simulink model "gravcomp"  (Simulink 7.5)
settings: Solver=ode3  StartTime=0.0  StopTime=inf  FixedStep=.002  RelTol=1e-3
values from neighbouring files (symbols this model uses):
  arm_home = [ -0.1106   -1.9490   -0.1920    3.1840 ]    [NEW_PID_4DOF.m]    (also in SetPoint_Control.m = [ -0.1106   -1.9490   -0.1920    3.1840    0.2825    0.0969 ; Stochastic_coriolis.m = [  -0.1106   -1.9490   -0.1920    3.1840    0.2825    0.0969; Untitled4.m = [ -0.1106   -1.9490   -0.1920    3.1840    0.2825    0.0969 )
undefined symbols (not defined in the file or in its folder): arm_j2mt, arm_m2jp, bit, CAN_init, enc_per_rev, fdesignblkfcn, FT_init, gcbh, hand_on, MT_init, puck_I_per_Nm, rotFT2Hand, sample_time, Standard, VL1_init, VL2_init
libraries: simulink x358, xpclib x28, xpcutilitieslib x6, dspmathops x1
(part 2 of 3)

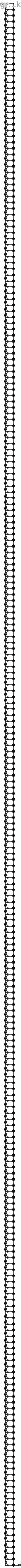
== system gravcomp/Get FT/Get Force Torque/New Filter/Generated Filter Block ==
  Input : Inport
  BodyDelay{2..260} (259 alike) : simulink/Discrete/Integer Delay  vinit=0  samptime=-1  NumDelays=1
  BodyLSum{2..260} (259 alike) : Sum  Inputs=++|  OutScaling=1  RndMeth=Nearest  SaturateOnIntegerOverflow=on  OutDataTypeStr=Inherit: Same as first input
  b(1) : Gain  Gain=0.00070417510961843762  ParameterDataTypeMode=Specify via dialog  ParameterDataType=float('double')  ParamDataTypeStr=float('double')  OutScaling=1  RndMeth=Nearest  SaturateOnIntegerOverflow=on  OutDataTypeStr=Inherit: Same as input
  b(10) : Gain  Gain=0.00065890295760926093  ParameterDataTypeMode=Specify via dialog  ParameterDataType=float('double')  ParamDataTypeStr=float('double')  OutScaling=1  RndMeth=Nearest  SaturateOnIntegerOverflow=on  OutDataTypeStr=Inherit: Same as input
  b(100) : Gain  Gain=0.0062955708769956709  ParameterDataTypeMode=Specify via dialog  ParameterDataType=float('double')  ParamDataTypeStr=float('double')  OutScaling=1  RndMeth=Nearest  SaturateOnIntegerOverflow=on  OutDataTypeStr=Inherit: Same as input
  b(101) : Gain  Gain=0.0071285779409714038  ParameterDataTypeMode=Specify via dialog  ParameterDataType=float('double')  ParamDataTypeStr=float('double')  OutScaling=1  RndMeth=Nearest  SaturateOnIntegerOverflow=on  OutDataTypeStr=Inherit: Same as input
  b(102) : Gain  Gain=0.0079758397591894736  ParameterDataTypeMode=Specify via dialog  ParameterDataType=float('double')  ParamDataTypeStr=float('double')  OutScaling=1  RndMeth=Nearest  SaturateOnIntegerOverflow=on  OutDataTypeStr=Inherit: Same as input
  b(103) : Gain  Gain=0.0088344622316554079  ParameterDataTypeMode=Specify via dialog  ParameterDataType=float('double')  ParamDataTypeStr=float('double')  OutScaling=1  RndMeth=Nearest  SaturateOnIntegerOverflow=on  OutDataTypeStr=Inherit: Same as input
  b(104) : Gain  Gain=0.0097014714889568053  ParameterDataTypeMode=Specify via dialog  ParameterDataType=float('double')  ParamDataTypeStr=float('double')  OutScaling=1  RndMeth=Nearest  SaturateOnIntegerOverflow=on  OutDataTypeStr=Inherit: Same as input
  b(105) : Gain  Gain=0.010573811729065394  ParameterDataTypeMode=Specify via dialog  ParameterDataType=float('double')  ParamDataTypeStr=float('double')  OutScaling=1  RndMeth=Nearest  SaturateOnIntegerOverflow=on  OutDataTypeStr=Inherit: Same as input
  b(106) : Gain  Gain=0.011448280041578808  ParameterDataTypeMode=Specify via dialog  ParameterDataType=float('double')  ParamDataTypeStr=float('double')  OutScaling=1  RndMeth=Nearest  SaturateOnIntegerOverflow=on  OutDataTypeStr=Inherit: Same as input
  b(107) : Gain  Gain=0.012321705260453951  ParameterDataTypeMode=Specify via dialog  ParameterDataType=float('double')  ParamDataTypeStr=float('double')  OutScaling=1  RndMeth=Nearest  SaturateOnIntegerOverflow=on  OutDataTypeStr=Inherit: Same as input
  b(108) : Gain  Gain=0.01319080449047489  ParameterDataTypeMode=Specify via dialog  ParameterDataType=float('double')  ParamDataTypeStr=float('double')  OutScaling=1  RndMeth=Nearest  SaturateOnIntegerOverflow=on  OutDataTypeStr=Inherit: Same as input
  b(109) : Gain  Gain=0.014052286654709126  ParameterDataTypeMode=Specify via dialog  ParameterDataType=float('double')  ParamDataTypeStr=float('double')  OutScaling=1  RndMeth=Nearest  SaturateOnIntegerOverflow=on  OutDataTypeStr=Inherit: Same as input
  b(11) : Gain  Gain=0.00072315700075571872  ParameterDataTypeMode=Specify via dialog  ParameterDataType=float('double')  ParamDataTypeStr=float('double')  OutScaling=1  RndMeth=Nearest  SaturateOnIntegerOverflow=on  OutDataTypeStr=Inherit: Same as input
  b(110) : Gain  Gain=0.014902829506351663  ParameterDataTypeMode=Specify via dialog  ParameterDataType=float('double')  ParamDataTypeStr=float('double')  OutScaling=1  RndMeth=Nearest  SaturateOnIntegerOverflow=on  OutDataTypeStr=Inherit: Same as input
  b(111) : Gain  Gain=0.015739153848427601  ParameterDataTypeMode=Specify via dialog  ParameterDataType=float('double')  ParamDataTypeStr=float('double')  OutScaling=1  RndMeth=Nearest  SaturateOnIntegerOverflow=on  OutDataTypeStr=Inherit: Same as input
  b(112) : Gain  Gain=0.016557936832079102  ParameterDataTypeMode=Specify via dialog  ParameterDataType=float('double')  ParamDataTypeStr=float('double')  OutScaling=1  RndMeth=Nearest  SaturateOnIntegerOverflow=on  OutDataTypeStr=Inherit: Same as input
  b(113) : Gain  Gain=0.017355946398475892  ParameterDataTypeMode=Specify via dialog  ParameterDataType=float('double')  ParamDataTypeStr=float('double')  OutScaling=1  RndMeth=Nearest  SaturateOnIntegerOverflow=on  OutDataTypeStr=Inherit: Same as input
  b(114) : Gain  Gain=0.018129972748423043  ParameterDataTypeMode=Specify via dialog  ParameterDataType=float('double')  ParamDataTypeStr=float('double')  OutScaling=1  RndMeth=Nearest  SaturateOnIntegerOverflow=on  OutDataTypeStr=Inherit: Same as input
  b(115) : Gain  Gain=0.018876872775595334  ParameterDataTypeMode=Specify via dialog  ParameterDataType=float('double')  ParamDataTypeStr=float('double')  OutScaling=1  RndMeth=Nearest  SaturateOnIntegerOverflow=on  OutDataTypeStr=Inherit: Same as input
  b(116) : Gain  Gain=0.01959360140160285  ParameterDataTypeMode=Specify via dialog  ParameterDataType=float('double')  ParamDataTypeStr=float('double')  OutScaling=1  RndMeth=Nearest  SaturateOnIntegerOverflow=on  OutDataTypeStr=Inherit: Same as input
  b(117) : Gain  Gain=0.02027722646982065  ParameterDataTypeMode=Specify via dialog  ParameterDataType=float('double')  ParamDataTypeStr=float('double')  OutScaling=1  RndMeth=Nearest  SaturateOnIntegerOverflow=on  OutDataTypeStr=Inherit: Same as input
  b(118) : Gain  Gain=0.020924875790597104  ParameterDataTypeMode=Specify via dialog  ParameterDataType=float('double')  ParamDataTypeStr=float('double')  OutScaling=1  RndMeth=Nearest  SaturateOnIntegerOverflow=on  OutDataTypeStr=Inherit: Same as input
  b(119) : Gain  Gain=0.021533887742310798  ParameterDataTypeMode=Specify via dialog  ParameterDataType=float('double')  ParamDataTypeStr=float('double')  OutScaling=1  RndMeth=Nearest  SaturateOnIntegerOverflow=on  OutDataTypeStr=Inherit: Same as input
  b(12) : Gain  Gain=0.00078945898775655888  ParameterDataTypeMode=Specify via dialog  ParameterDataType=float('double')  ParamDataTypeStr=float('double')  OutScaling=1  RndMeth=Nearest  SaturateOnIntegerOverflow=on  OutDataTypeStr=Inherit: Same as input
  b(120) : Gain  Gain=0.022101695679814737  ParameterDataTypeMode=Specify via dialog  ParameterDataType=float('double')  ParamDataTypeStr=float('double')  OutScaling=1  RndMeth=Nearest  SaturateOnIntegerOverflow=on  OutDataTypeStr=Inherit: Same as input
  b(121) : Gain  Gain=0.022625902042927921  ParameterDataTypeMode=Specify via dialog  ParameterDataType=float('double')  ParamDataTypeStr=float('double')  OutScaling=1  RndMeth=Nearest  SaturateOnIntegerOverflow=on  OutDataTypeStr=Inherit: Same as input
  b(122) : Gain  Gain=0.023104290316677902  ParameterDataTypeMode=Specify via dialog  ParameterDataType=float('double')  ParamDataTypeStr=float('double')  OutScaling=1  RndMeth=Nearest  SaturateOnIntegerOverflow=on  OutDataTypeStr=Inherit: Same as input
  b(123) : Gain  Gain=0.023534842993415066  ParameterDataTypeMode=Specify via dialog  ParameterDataType=float('double')  ParamDataTypeStr=float('double')  OutScaling=1  RndMeth=Nearest  SaturateOnIntegerOverflow=on  OutDataTypeStr=Inherit: Same as input
  b(124) : Gain  Gain=0.023915699194656088  ParameterDataTypeMode=Specify via dialog  ParameterDataType=float('double')  ParamDataTypeStr=float('double')  OutScaling=1  RndMeth=Nearest  SaturateOnIntegerOverflow=on  OutDataTypeStr=Inherit: Same as input
  b(125) : Gain  Gain=0.024245248888987846  ParameterDataTypeMode=Specify via dialog  ParameterDataType=float('double')  ParamDataTypeStr=float('double')  OutScaling=1  RndMeth=Nearest  SaturateOnIntegerOverflow=on  OutDataTypeStr=Inherit: Same as input
  b(126) : Gain  Gain=0.024522074604789321  ParameterDataTypeMode=Specify via dialog  ParameterDataType=float('double')  ParamDataTypeStr=float('double')  OutScaling=1  RndMeth=Nearest  SaturateOnIntegerOverflow=on  OutDataTypeStr=Inherit: Same as input
  b(127) : Gain  Gain=0.024744974417626367  ParameterDataTypeMode=Specify via dialog  ParameterDataType=float('double')  ParamDataTypeStr=float('double')  OutScaling=1  RndMeth=Nearest  SaturateOnIntegerOverflow=on  OutDataTypeStr=Inherit: Same as input
  b(128) : Gain  Gain=0.024913000551013219  ParameterDataTypeMode=Specify via dialog  ParameterDataType=float('double')  ParamDataTypeStr=float('double')  OutScaling=1  RndMeth=Nearest  SaturateOnIntegerOverflow=on  OutDataTypeStr=Inherit: Same as input
  b(129) : Gain  Gain=0.025025430343517754  ParameterDataTypeMode=Specify via dialog  ParameterDataType=float('double')  ParamDataTypeStr=float('double')  OutScaling=1  RndMeth=Nearest  SaturateOnIntegerOverflow=on  OutDataTypeStr=Inherit: Same as input
  b(13) : Gain  Gain=0.00085906126191019659  ParameterDataTypeMode=Specify via dialog  ParameterDataType=float('double')  ParamDataTypeStr=float('double')  OutScaling=1  RndMeth=Nearest  SaturateOnIntegerOverflow=on  OutDataTypeStr=Inherit: Same as input
  b(130) : Gain  Gain=0.025081755990063945  ParameterDataTypeMode=Specify via dialog  ParameterDataType=float('double')  ParamDataTypeStr=float('double')  OutScaling=1  RndMeth=Nearest  SaturateOnIntegerOverflow=on  OutDataTypeStr=Inherit: Same as input
  b(131) : Gain  Gain=0.025081755990063945  ParameterDataTypeMode=Specify via dialog  ParameterDataType=float('double')  ParamDataTypeStr=float('double')  OutScaling=1  RndMeth=Nearest  SaturateOnIntegerOverflow=on  OutDataTypeStr=Inherit: Same as input
  b(132) : Gain  Gain=0.025025430343517754  ParameterDataTypeMode=Specify via dialog  ParameterDataType=float('double')  ParamDataTypeStr=float('double')  OutScaling=1  RndMeth=Nearest  SaturateOnIntegerOverflow=on  OutDataTypeStr=Inherit: Same as input
  b(133) : Gain  Gain=0.024913000551013219  ParameterDataTypeMode=Specify via dialog  ParameterDataType=float('double')  ParamDataTypeStr=float('double')  OutScaling=1  RndMeth=Nearest  SaturateOnIntegerOverflow=on  OutDataTypeStr=Inherit: Same as input
  b(134) : Gain  Gain=0.024744974417626367  ParameterDataTypeMode=Specify via dialog  ParameterDataType=float('double')  ParamDataTypeStr=float('double')  OutScaling=1  RndMeth=Nearest  SaturateOnIntegerOverflow=on  OutDataTypeStr=Inherit: Same as input
  b(135) : Gain  Gain=0.024522074604789321  ParameterDataTypeMode=Specify via dialog  ParameterDataType=float('double')  ParamDataTypeStr=float('double')  OutScaling=1  RndMeth=Nearest  SaturateOnIntegerOverflow=on  OutDataTypeStr=Inherit: Same as input
  b(136) : Gain  Gain=0.024245248888987846  ParameterDataTypeMode=Specify via dialog  ParameterDataType=float('double')  ParamDataTypeStr=float('double')  OutScaling=1  RndMeth=Nearest  SaturateOnIntegerOverflow=on  OutDataTypeStr=Inherit: Same as input
  b(137) : Gain  Gain=0.023915699194656088  ParameterDataTypeMode=Specify via dialog  ParameterDataType=float('double')  ParamDataTypeStr=float('double')  OutScaling=1  RndMeth=Nearest  SaturateOnIntegerOverflow=on  OutDataTypeStr=Inherit: Same as input
  b(138) : Gain  Gain=0.023534842993415066  ParameterDataTypeMode=Specify via dialog  ParameterDataType=float('double')  ParamDataTypeStr=float('double')  OutScaling=1  RndMeth=Nearest  SaturateOnIntegerOverflow=on  OutDataTypeStr=Inherit: Same as input
  b(139) : Gain  Gain=0.023104290316677902  ParameterDataTypeMode=Specify via dialog  ParameterDataType=float('double')  ParamDataTypeStr=float('double')  OutScaling=1  RndMeth=Nearest  SaturateOnIntegerOverflow=on  OutDataTypeStr=Inherit: Same as input
  b(14) : Gain  Gain=0.000928205688470267  ParameterDataTypeMode=Specify via dialog  ParameterDataType=float('double')  ParamDataTypeStr=float('double')  OutScaling=1  RndMeth=Nearest  SaturateOnIntegerOverflow=on  OutDataTypeStr=Inherit: Same as input
  b(140) : Gain  Gain=0.022625902042927921  ParameterDataTypeMode=Specify via dialog  ParameterDataType=float('double')  ParamDataTypeStr=float('double')  OutScaling=1  RndMeth=Nearest  SaturateOnIntegerOverflow=on  OutDataTypeStr=Inherit: Same as input
  b(141) : Gain  Gain=0.022101695679814737  ParameterDataTypeMode=Specify via dialog  ParameterDataType=float('double')  ParamDataTypeStr=float('double')  OutScaling=1  RndMeth=Nearest  SaturateOnIntegerOverflow=on  OutDataTypeStr=Inherit: Same as input
  b(142) : Gain  Gain=0.021533887742310798  ParameterDataTypeMode=Specify via dialog  ParameterDataType=float('double')  ParamDataTypeStr=float('double')  OutScaling=1  RndMeth=Nearest  SaturateOnIntegerOverflow=on  OutDataTypeStr=Inherit: Same as input
  b(143) : Gain  Gain=0.020924875790597104  ParameterDataTypeMode=Specify via dialog  ParameterDataType=float('double')  ParamDataTypeStr=float('double')  OutScaling=1  RndMeth=Nearest  SaturateOnIntegerOverflow=on  OutDataTypeStr=Inherit: Same as input
  b(144) : Gain  Gain=0.02027722646982065  ParameterDataTypeMode=Specify via dialog  ParameterDataType=float('double')  ParamDataTypeStr=float('double')  OutScaling=1  RndMeth=Nearest  SaturateOnIntegerOverflow=on  OutDataTypeStr=Inherit: Same as input
  b(145) : Gain  Gain=0.01959360140160285  ParameterDataTypeMode=Specify via dialog  ParameterDataType=float('double')  ParamDataTypeStr=float('double')  OutScaling=1  RndMeth=Nearest  SaturateOnIntegerOverflow=on  OutDataTypeStr=Inherit: Same as input
  b(146) : Gain  Gain=0.018876872775595334  ParameterDataTypeMode=Specify via dialog  ParameterDataType=float('double')  ParamDataTypeStr=float('double')  OutScaling=1  RndMeth=Nearest  SaturateOnIntegerOverflow=on  OutDataTypeStr=Inherit: Same as input
  b(147) : Gain  Gain=0.018129972748423043  ParameterDataTypeMode=Specify via dialog  ParameterDataType=float('double')  ParamDataTypeStr=float('double')  OutScaling=1  RndMeth=Nearest  SaturateOnIntegerOverflow=on  OutDataTypeStr=Inherit: Same as input
  b(148) : Gain  Gain=0.017355946398475892  ParameterDataTypeMode=Specify via dialog  ParameterDataType=float('double')  ParamDataTypeStr=float('double')  OutScaling=1  RndMeth=Nearest  SaturateOnIntegerOverflow=on  OutDataTypeStr=Inherit: Same as input
  b(149) : Gain  Gain=0.016557936832079102  ParameterDataTypeMode=Specify via dialog  ParameterDataType=float('double')  ParamDataTypeStr=float('double')  OutScaling=1  RndMeth=Nearest  SaturateOnIntegerOverflow=on  OutDataTypeStr=Inherit: Same as input
  b(15) : Gain  Gain=0.00099957917679242272  ParameterDataTypeMode=Specify via dialog  ParameterDataType=float('double')  ParamDataTypeStr=float('double')  OutScaling=1  RndMeth=Nearest  SaturateOnIntegerOverflow=on  OutDataTypeStr=Inherit: Same as input
  b(150) : Gain  Gain=0.015739153848427601  ParameterDataTypeMode=Specify via dialog  ParameterDataType=float('double')  ParamDataTypeStr=float('double')  OutScaling=1  RndMeth=Nearest  SaturateOnIntegerOverflow=on  OutDataTypeStr=Inherit: Same as input
  b(151) : Gain  Gain=0.014902829506351663  ParameterDataTypeMode=Specify via dialog  ParameterDataType=float('double')  ParamDataTypeStr=float('double')  OutScaling=1  RndMeth=Nearest  SaturateOnIntegerOverflow=on  OutDataTypeStr=Inherit: Same as input
  b(152) : Gain  Gain=0.014052286654709126  ParameterDataTypeMode=Specify via dialog  ParameterDataType=float('double')  ParamDataTypeStr=float('double')  OutScaling=1  RndMeth=Nearest  SaturateOnIntegerOverflow=on  OutDataTypeStr=Inherit: Same as input
  b(153) : Gain  Gain=0.01319080449047489  ParameterDataTypeMode=Specify via dialog  ParameterDataType=float('double')  ParamDataTypeStr=float('double')  OutScaling=1  RndMeth=Nearest  SaturateOnIntegerOverflow=on  OutDataTypeStr=Inherit: Same as input
  b(154) : Gain  Gain=0.012321705260453951  ParameterDataTypeMode=Specify via dialog  ParameterDataType=float('double')  ParamDataTypeStr=float('double')  OutScaling=1  RndMeth=Nearest  SaturateOnIntegerOverflow=on  OutDataTypeStr=Inherit: Same as input
  b(155) : Gain  Gain=0.011448280041578808  ParameterDataTypeMode=Specify via dialog  ParameterDataType=float('double')  ParamDataTypeStr=float('double')  OutScaling=1  RndMeth=Nearest  SaturateOnIntegerOverflow=on  OutDataTypeStr=Inherit: Same as input
  b(156) : Gain  Gain=0.010573811729065394  ParameterDataTypeMode=Specify via dialog  ParameterDataType=float('double')  ParamDataTypeStr=float('double')  OutScaling=1  RndMeth=Nearest  SaturateOnIntegerOverflow=on  OutDataTypeStr=Inherit: Same as input
  b(157) : Gain  Gain=0.0097014714889568053  ParameterDataTypeMode=Specify via dialog  ParameterDataType=float('double')  ParamDataTypeStr=float('double')  OutScaling=1  RndMeth=Nearest  SaturateOnIntegerOverflow=on  OutDataTypeStr=Inherit: Same as input
  b(158) : Gain  Gain=0.0088344622316554079  ParameterDataTypeMode=Specify via dialog  ParameterDataType=float('double')  ParamDataTypeStr=float('double')  OutScaling=1  RndMeth=Nearest  SaturateOnIntegerOverflow=on  OutDataTypeStr=Inherit: Same as input
  b(159) : Gain  Gain=0.0079758397591894736  ParameterDataTypeMode=Specify via dialog  ParameterDataType=float('double')  ParamDataTypeStr=float('double')  OutScaling=1  RndMeth=Nearest  SaturateOnIntegerOverflow=on  OutDataTypeStr=Inherit: Same as input
  b(16) : Gain  Gain=0.0010715809286023286  ParameterDataTypeMode=Specify via dialog  ParameterDataType=float('double')  ParamDataTypeStr=float('double')  OutScaling=1  RndMeth=Nearest  SaturateOnIntegerOverflow=on  OutDataTypeStr=Inherit: Same as input
  b(160) : Gain  Gain=0.0071285779409714038  ParameterDataTypeMode=Specify via dialog  ParameterDataType=float('double')  ParamDataTypeStr=float('double')  OutScaling=1  RndMeth=Nearest  SaturateOnIntegerOverflow=on  OutDataTypeStr=Inherit: Same as input
  b(161) : Gain  Gain=0.0062955708769956709  ParameterDataTypeMode=Specify via dialog  ParameterDataType=float('double')  ParamDataTypeStr=float('double')  OutScaling=1  RndMeth=Nearest  SaturateOnIntegerOverflow=on  OutDataTypeStr=Inherit: Same as input
  b(162) : Gain  Gain=0.0054795719185856736  ParameterDataTypeMode=Specify via dialog  ParameterDataType=float('double')  ParamDataTypeStr=float('double')  OutScaling=1  RndMeth=Nearest  SaturateOnIntegerOverflow=on  OutDataTypeStr=Inherit: Same as input
  b(163) : Gain  Gain=0.0046831909839310645  ParameterDataTypeMode=Specify via dialog  ParameterDataType=float('double')  ParamDataTypeStr=float('double')  OutScaling=1  RndMeth=Nearest  SaturateOnIntegerOverflow=on  OutDataTypeStr=Inherit: Same as input
  b(164) : Gain  Gain=0.003908939056141314  ParameterDataTypeMode=Specify via dialog  ParameterDataType=float('double')  ParamDataTypeStr=float('double')  OutScaling=1  RndMeth=Nearest  SaturateOnIntegerOverflow=on  OutDataTypeStr=Inherit: Same as input
  b(165) : Gain  Gain=0.0031591101868804696  ParameterDataTypeMode=Specify via dialog  ParameterDataType=float('double')  ParamDataTypeStr=float('double')  OutScaling=1  RndMeth=Nearest  SaturateOnIntegerOverflow=on  OutDataTypeStr=Inherit: Same as input
  b(166) : Gain  Gain=0.0024358839160543953  ParameterDataTypeMode=Specify via dialog  ParameterDataType=float('double')  ParamDataTypeStr=float('double')  OutScaling=1  RndMeth=Nearest  SaturateOnIntegerOverflow=on  OutDataTypeStr=Inherit: Same as input
  b(167) : Gain  Gain=0.0017412535010850488  ParameterDataTypeMode=Specify via dialog  ParameterDataType=float('double')  ParamDataTypeStr=float('double')  OutScaling=1  RndMeth=Nearest  SaturateOnIntegerOverflow=on  OutDataTypeStr=Inherit: Same as input
  b(168) : Gain  Gain=0.0010770433381879106  ParameterDataTypeMode=Specify via dialog  ParameterDataType=float('double')  ParamDataTypeStr=float('double')  OutScaling=1  RndMeth=Nearest  SaturateOnIntegerOverflow=on  OutDataTypeStr=Inherit: Same as input
  b(169) : Gain  Gain=0.00044484680086729451  ParameterDataTypeMode=Specify via dialog  ParameterDataType=float('double')  ParamDataTypeStr=float('double')  OutScaling=1  RndMeth=Nearest  SaturateOnIntegerOverflow=on  OutDataTypeStr=Inherit: Same as input
  b(17) : Gain  Gain=0.0011435663265835921  ParameterDataTypeMode=Specify via dialog  ParameterDataType=float('double')  ParamDataTypeStr=float('double')  OutScaling=1  RndMeth=Nearest  SaturateOnIntegerOverflow=on  OutDataTypeStr=Inherit: Same as input
  b(170) : Gain  Gain=-0.00015384920636331843  ParameterDataTypeMode=Specify via dialog  ParameterDataType=float('double')  ParamDataTypeStr=float('double')  OutScaling=1  RndMeth=Nearest  SaturateOnIntegerOverflow=on  OutDataTypeStr=Inherit: Same as input
  b(171) : Gain  Gain=-0.00071779930929411525  ParameterDataTypeMode=Specify via dialog  ParameterDataType=float('double')  ParamDataTypeStr=float('double')  OutScaling=1  RndMeth=Nearest  SaturateOnIntegerOverflow=on  OutDataTypeStr=Inherit: Same as input
  b(172) : Gain  Gain=-0.0012459755928315391  ParameterDataTypeMode=Specify via dialog  ParameterDataType=float('double')  ParamDataTypeStr=float('double')  OutScaling=1  RndMeth=Nearest  SaturateOnIntegerOverflow=on  OutDataTypeStr=Inherit: Same as input
  b(173) : Gain  Gain=-0.0017374680097337761  ParameterDataTypeMode=Specify via dialog  ParameterDataType=float('double')  ParamDataTypeStr=float('double')  OutScaling=1  RndMeth=Nearest  SaturateOnIntegerOverflow=on  OutDataTypeStr=Inherit: Same as input
  b(174) : Gain  Gain=-0.0021916374965953132  ParameterDataTypeMode=Specify via dialog  ParameterDataType=float('double')  ParamDataTypeStr=float('double')  OutScaling=1  RndMeth=Nearest  SaturateOnIntegerOverflow=on  OutDataTypeStr=Inherit: Same as input
  b(175) : Gain  Gain=-0.0026079964847781222  ParameterDataTypeMode=Specify via dialog  ParameterDataType=float('double')  ParamDataTypeStr=float('double')  OutScaling=1  RndMeth=Nearest  SaturateOnIntegerOverflow=on  OutDataTypeStr=Inherit: Same as input
  b(176) : Gain  Gain=-0.0029862469165041388  ParameterDataTypeMode=Specify via dialog  ParameterDataType=float('double')  ParamDataTypeStr=float('double')  OutScaling=1  RndMeth=Nearest  SaturateOnIntegerOverflow=on  OutDataTypeStr=Inherit: Same as input
  b(177) : Gain  Gain=-0.0033263178221817377  ParameterDataTypeMode=Specify via dialog  ParameterDataType=float('double')  ParamDataTypeStr=float('double')  OutScaling=1  RndMeth=Nearest  SaturateOnIntegerOverflow=on  OutDataTypeStr=Inherit: Same as input
  b(178) : Gain  Gain=-0.0036282918249470573  ParameterDataTypeMode=Specify via dialog  ParameterDataType=float('double')  ParamDataTypeStr=float('double')  OutScaling=1  RndMeth=Nearest  SaturateOnIntegerOverflow=on  OutDataTypeStr=Inherit: Same as input
  b(179) : Gain  Gain=-0.0038924172738207274  ParameterDataTypeMode=Specify via dialog  ParameterDataType=float('double')  ParamDataTypeStr=float('double')  OutScaling=1  RndMeth=Nearest  SaturateOnIntegerOverflow=on  OutDataTypeStr=Inherit: Same as input
  b(18) : Gain  Gain=0.001215524986978665  ParameterDataTypeMode=Specify via dialog  ParameterDataType=float('double')  ParamDataTypeStr=float('double')  OutScaling=1  RndMeth=Nearest  SaturateOnIntegerOverflow=on  OutDataTypeStr=Inherit: Same as input
  b(180) : Gain  Gain=-0.0041191558942448771  ParameterDataTypeMode=Specify via dialog  ParameterDataType=float('double')  ParamDataTypeStr=float('double')  OutScaling=1  RndMeth=Nearest  SaturateOnIntegerOverflow=on  OutDataTypeStr=Inherit: Same as input
  b(181) : Gain  Gain=-0.0043091320843662781  ParameterDataTypeMode=Specify via dialog  ParameterDataType=float('double')  ParamDataTypeStr=float('double')  OutScaling=1  RndMeth=Nearest  SaturateOnIntegerOverflow=on  OutDataTypeStr=Inherit: Same as input
  b(182) : Gain  Gain=-0.0044630950959934825  ParameterDataTypeMode=Specify via dialog  ParameterDataType=float('double')  ParamDataTypeStr=float('double')  OutScaling=1  RndMeth=Nearest  SaturateOnIntegerOverflow=on  OutDataTypeStr=Inherit: Same as input
  b(183) : Gain  Gain=-0.0045819428812625337  ParameterDataTypeMode=Specify via dialog  ParameterDataType=float('double')  ParamDataTypeStr=float('double')  OutScaling=1  RndMeth=Nearest  SaturateOnIntegerOverflow=on  OutDataTypeStr=Inherit: Same as input
  b(184) : Gain  Gain=-0.0046668113226438135  ParameterDataTypeMode=Specify via dialog  ParameterDataType=float('double')  ParamDataTypeStr=float('double')  OutScaling=1  RndMeth=Nearest  SaturateOnIntegerOverflow=on  OutDataTypeStr=Inherit: Same as input
  b(185) : Gain  Gain=-0.0047188020939299127  ParameterDataTypeMode=Specify via dialog  ParameterDataType=float('double')  ParamDataTypeStr=float('double')  OutScaling=1  RndMeth=Nearest  SaturateOnIntegerOverflow=on  OutDataTypeStr=Inherit: Same as input
  b(186) : Gain  Gain=-0.0047393103130561991  ParameterDataTypeMode=Specify via dialog  ParameterDataType=float('double')  ParamDataTypeStr=float('double')  OutScaling=1  RndMeth=Nearest  SaturateOnIntegerOverflow=on  OutDataTypeStr=Inherit: Same as input
  b(187) : Gain  Gain=-0.0047297082884658788  ParameterDataTypeMode=Specify via dialog  ParameterDataType=float('double')  ParamDataTypeStr=float('double')  OutScaling=1  RndMeth=Nearest  SaturateOnIntegerOverflow=on  OutDataTypeStr=Inherit: Same as input
  b(188) : Gain  Gain=-0.0046915387161280356  ParameterDataTypeMode=Specify via dialog  ParameterDataType=float('double')  ParamDataTypeStr=float('double')  OutScaling=1  RndMeth=Nearest  SaturateOnIntegerOverflow=on  OutDataTypeStr=Inherit: Same as input
  b(189) : Gain  Gain=-0.0046264252289973861  ParameterDataTypeMode=Specify via dialog  ParameterDataType=float('double')  ParamDataTypeStr=float('double')  OutScaling=1  RndMeth=Nearest  SaturateOnIntegerOverflow=on  OutDataTypeStr=Inherit: Same as input
  b(19) : Gain  Gain=0.0012865512850236843  ParameterDataTypeMode=Specify via dialog  ParameterDataType=float('double')  ParamDataTypeStr=float('double')  OutScaling=1  RndMeth=Nearest  SaturateOnIntegerOverflow=on  OutDataTypeStr=Inherit: Same as input
  b(190) : Gain  Gain=-0.004536068879832213  ParameterDataTypeMode=Specify via dialog  ParameterDataType=float('double')  ParamDataTypeStr=float('double')  OutScaling=1  RndMeth=Nearest  SaturateOnIntegerOverflow=on  OutDataTypeStr=Inherit: Same as input
  b(191) : Gain  Gain=-0.0044221700763802108  ParameterDataTypeMode=Specify via dialog  ParameterDataType=float('double')  ParamDataTypeStr=float('double')  OutScaling=1  RndMeth=Nearest  SaturateOnIntegerOverflow=on  OutDataTypeStr=Inherit: Same as input
  b(192) : Gain  Gain=-0.0042865991428804734  ParameterDataTypeMode=Specify via dialog  ParameterDataType=float('double')  ParamDataTypeStr=float('double')  OutScaling=1  RndMeth=Nearest  SaturateOnIntegerOverflow=on  OutDataTypeStr=Inherit: Same as input
  b(193) : Gain  Gain=-0.0041311777625552227  ParameterDataTypeMode=Specify via dialog  ParameterDataType=float('double')  ParamDataTypeStr=float('double')  OutScaling=1  RndMeth=Nearest  SaturateOnIntegerOverflow=on  OutDataTypeStr=Inherit: Same as input
  b(194) : Gain  Gain=-0.0039577961713118419  ParameterDataTypeMode=Specify via dialog  ParameterDataType=float('double')  ParamDataTypeStr=float('double')  OutScaling=1  RndMeth=Nearest  SaturateOnIntegerOverflow=on  OutDataTypeStr=Inherit: Same as input
  b(195) : Gain  Gain=-0.0037682781895092285  ParameterDataTypeMode=Specify via dialog  ParameterDataType=float('double')  ParamDataTypeStr=float('double')  OutScaling=1  RndMeth=Nearest  SaturateOnIntegerOverflow=on  OutDataTypeStr=Inherit: Same as input
  b(196) : Gain  Gain=-0.0035646528383071309  ParameterDataTypeMode=Specify via dialog  ParameterDataType=float('double')  ParamDataTypeStr=float('double')  OutScaling=1  RndMeth=Nearest  SaturateOnIntegerOverflow=on  OutDataTypeStr=Inherit: Same as input
  b(197) : Gain  Gain=-0.0033486524967329487  ParameterDataTypeMode=Specify via dialog  ParameterDataType=float('double')  ParamDataTypeStr=float('double')  OutScaling=1  RndMeth=Nearest  SaturateOnIntegerOverflow=on  OutDataTypeStr=Inherit: Same as input
  b(198) : Gain  Gain=-0.0031222962030929349  ParameterDataTypeMode=Specify via dialog  ParameterDataType=float('double')  ParamDataTypeStr=float('double')  OutScaling=1  RndMeth=Nearest  SaturateOnIntegerOverflow=on  OutDataTypeStr=Inherit: Same as input
  b(199) : Gain  Gain=-0.0028873200222469617  ParameterDataTypeMode=Specify via dialog  ParameterDataType=float('double')  ParamDataTypeStr=float('double')  OutScaling=1  RndMeth=Nearest  SaturateOnIntegerOverflow=on  OutDataTypeStr=Inherit: Same as input
  b(2) : Gain  Gain=0.00024423156750045524  ParameterDataTypeMode=Specify via dialog  ParameterDataType=float('double')  ParamDataTypeStr=float('double')  OutScaling=1  RndMeth=Nearest  SaturateOnIntegerOverflow=on  OutDataTypeStr=Inherit: Same as input
  b(20) : Gain  Gain=0.0013564706827517313  ParameterDataTypeMode=Specify via dialog  ParameterDataType=float('double')  ParamDataTypeStr=float('double')  OutScaling=1  RndMeth=Nearest  SaturateOnIntegerOverflow=on  OutDataTypeStr=Inherit: Same as input
  b(200) : Gain  Gain=-0.0026455884436352908  ParameterDataTypeMode=Specify via dialog  ParameterDataType=float('double')  ParamDataTypeStr=float('double')  OutScaling=1  RndMeth=Nearest  SaturateOnIntegerOverflow=on  OutDataTypeStr=Inherit: Same as input
  b(201) : Gain  Gain=-0.0023988698157260263  ParameterDataTypeMode=Specify via dialog  ParameterDataType=float('double')  ParamDataTypeStr=float('double')  OutScaling=1  RndMeth=Nearest  SaturateOnIntegerOverflow=on  OutDataTypeStr=Inherit: Same as input
  b(202) : Gain  Gain=-0.002148902815176169  ParameterDataTypeMode=Specify via dialog  ParameterDataType=float('double')  ParamDataTypeStr=float('double')  OutScaling=1  RndMeth=Nearest  SaturateOnIntegerOverflow=on  OutDataTypeStr=Inherit: Same as input
  b(203) : Gain  Gain=-0.0018972524976453848  ParameterDataTypeMode=Specify via dialog  ParameterDataType=float('double')  ParamDataTypeStr=float('double')  OutScaling=1  RndMeth=Nearest  SaturateOnIntegerOverflow=on  OutDataTypeStr=Inherit: Same as input
  b(204) : Gain  Gain=-0.0016456276040868589  ParameterDataTypeMode=Specify via dialog  ParameterDataType=float('double')  ParamDataTypeStr=float('double')  OutScaling=1  RndMeth=Nearest  SaturateOnIntegerOverflow=on  OutDataTypeStr=Inherit: Same as input
  b(205) : Gain  Gain=-0.0013954701655563839  ParameterDataTypeMode=Specify via dialog  ParameterDataType=float('double')  ParamDataTypeStr=float('double')  OutScaling=1  RndMeth=Nearest  SaturateOnIntegerOverflow=on  OutDataTypeStr=Inherit: Same as input
  b(206) : Gain  Gain=-0.0011482695116857549  ParameterDataTypeMode=Specify via dialog  ParameterDataType=float('double')  ParamDataTypeStr=float('double')  OutScaling=1  RndMeth=Nearest  SaturateOnIntegerOverflow=on  OutDataTypeStr=Inherit: Same as input
  b(207) : Gain  Gain=-0.0009052529655871384  ParameterDataTypeMode=Specify via dialog  ParameterDataType=float('double')  ParamDataTypeStr=float('double')  OutScaling=1  RndMeth=Nearest  SaturateOnIntegerOverflow=on  OutDataTypeStr=Inherit: Same as input
  b(208) : Gain  Gain=-0.00066787760762591962  ParameterDataTypeMode=Specify via dialog  ParameterDataType=float('double')  ParamDataTypeStr=float('double')  OutScaling=1  RndMeth=Nearest  SaturateOnIntegerOverflow=on  OutDataTypeStr=Inherit: Same as input
  b(209) : Gain  Gain=-0.00043706573064342683  ParameterDataTypeMode=Specify via dialog  ParameterDataType=float('double')  ParamDataTypeStr=float('double')  OutScaling=1  RndMeth=Nearest  SaturateOnIntegerOverflow=on  OutDataTypeStr=Inherit: Same as input
  b(21) : Gain  Gain=0.0014245835558915126  ParameterDataTypeMode=Specify via dialog  ParameterDataType=float('double')  ParamDataTypeStr=float('double')  OutScaling=1  RndMeth=Nearest  SaturateOnIntegerOverflow=on  OutDataTypeStr=Inherit: Same as input
  b(210) : Gain  Gain=-0.00021409722155803576  ParameterDataTypeMode=Specify via dialog  ParameterDataType=float('double')  ParamDataTypeStr=float('double')  OutScaling=1  RndMeth=Nearest  SaturateOnIntegerOverflow=on  OutDataTypeStr=Inherit: Same as input
  b(211) : Gain  Gain=2.4895367239561282e-007  ParameterDataTypeMode=Specify via dialog  ParameterDataType=float('double')  ParamDataTypeStr=float('double')  OutScaling=1  RndMeth=Nearest  SaturateOnIntegerOverflow=on  OutDataTypeStr=Inherit: Same as input
  b(212) : Gain  Gain=0.00020504503595217299  ParameterDataTypeMode=Specify via dialog  ParameterDataType=float('double')  ParamDataTypeStr=float('double')  OutScaling=1  RndMeth=Nearest  SaturateOnIntegerOverflow=on  OutDataTypeStr=Inherit: Same as input
  b(213) : Gain  Gain=0.00039951833019874391  ParameterDataTypeMode=Specify via dialog  ParameterDataType=float('double')  ParamDataTypeStr=float('double')  OutScaling=1  RndMeth=Nearest  SaturateOnIntegerOverflow=on  OutDataTypeStr=Inherit: Same as input
  b(214) : Gain  Gain=0.00058302352831076721  ParameterDataTypeMode=Specify via dialog  ParameterDataType=float('double')  ParamDataTypeStr=float('double')  OutScaling=1  RndMeth=Nearest  SaturateOnIntegerOverflow=on  OutDataTypeStr=Inherit: Same as input
  b(215) : Gain  Gain=0.00075512721901295162  ParameterDataTypeMode=Specify via dialog  ParameterDataType=float('double')  ParamDataTypeStr=float('double')  OutScaling=1  RndMeth=Nearest  SaturateOnIntegerOverflow=on  OutDataTypeStr=Inherit: Same as input
  b(216) : Gain  Gain=0.00091520468672270927  ParameterDataTypeMode=Specify via dialog  ParameterDataType=float('double')  ParamDataTypeStr=float('double')  OutScaling=1  RndMeth=Nearest  SaturateOnIntegerOverflow=on  OutDataTypeStr=Inherit: Same as input
  b(217) : Gain  Gain=0.001063020174163772  ParameterDataTypeMode=Specify via dialog  ParameterDataType=float('double')  ParamDataTypeStr=float('double')  OutScaling=1  RndMeth=Nearest  SaturateOnIntegerOverflow=on  OutDataTypeStr=Inherit: Same as input
  b(218) : Gain  Gain=0.0011982302848979744  ParameterDataTypeMode=Specify via dialog  ParameterDataType=float('double')  ParamDataTypeStr=float('double')  OutScaling=1  RndMeth=Nearest  SaturateOnIntegerOverflow=on  OutDataTypeStr=Inherit: Same as input
  b(219) : Gain  Gain=0.0013208346129694928  ParameterDataTypeMode=Specify via dialog  ParameterDataType=float('double')  ParamDataTypeStr=float('double')  OutScaling=1  RndMeth=Nearest  SaturateOnIntegerOverflow=on  OutDataTypeStr=Inherit: Same as input
  b(22) : Gain  Gain=0.0014902408540535053  ParameterDataTypeMode=Specify via dialog  ParameterDataType=float('double')  ParamDataTypeStr=float('double')  OutScaling=1  RndMeth=Nearest  SaturateOnIntegerOverflow=on  OutDataTypeStr=Inherit: Same as input
  b(220) : Gain  Gain=0.001430483050405896  ParameterDataTypeMode=Specify via dialog  ParameterDataType=float('double')  ParamDataTypeStr=float('double')  OutScaling=1  RndMeth=Nearest  SaturateOnIntegerOverflow=on  OutDataTypeStr=Inherit: Same as input
  b(221) : Gain  Gain=0.0015275027261476678  ParameterDataTypeMode=Specify via dialog  ParameterDataType=float('double')  ParamDataTypeStr=float('double')  OutScaling=1  RndMeth=Nearest  SaturateOnIntegerOverflow=on  OutDataTypeStr=Inherit: Same as input
  b(222) : Gain  Gain=0.0016116862849141164  ParameterDataTypeMode=Specify via dialog  ParameterDataType=float('double')  ParamDataTypeStr=float('double')  OutScaling=1  RndMeth=Nearest  SaturateOnIntegerOverflow=on  OutDataTypeStr=Inherit: Same as input
  b(223) : Gain  Gain=0.0016834467566769996  ParameterDataTypeMode=Specify via dialog  ParameterDataType=float('double')  ParamDataTypeStr=float('double')  OutScaling=1  RndMeth=Nearest  SaturateOnIntegerOverflow=on  OutDataTypeStr=Inherit: Same as input
  b(224) : Gain  Gain=0.0017429852808810774  ParameterDataTypeMode=Specify via dialog  ParameterDataType=float('double')  ParamDataTypeStr=float('double')  OutScaling=1  RndMeth=Nearest  SaturateOnIntegerOverflow=on  OutDataTypeStr=Inherit: Same as input
  b(225) : Gain  Gain=0.0017904755880180506  ParameterDataTypeMode=Specify via dialog  ParameterDataType=float('double')  ParamDataTypeStr=float('double')  OutScaling=1  RndMeth=Nearest  SaturateOnIntegerOverflow=on  OutDataTypeStr=Inherit: Same as input
  b(226) : Gain  Gain=0.0018264374579876998  ParameterDataTypeMode=Specify via dialog  ParameterDataType=float('double')  ParamDataTypeStr=float('double')  OutScaling=1  RndMeth=Nearest  SaturateOnIntegerOverflow=on  OutDataTypeStr=Inherit: Same as input
  b(227) : Gain  Gain=0.0018513900016270467  ParameterDataTypeMode=Specify via dialog  ParameterDataType=float('double')  ParamDataTypeStr=float('double')  OutScaling=1  RndMeth=Nearest  SaturateOnIntegerOverflow=on  OutDataTypeStr=Inherit: Same as input
  b(228) : Gain  Gain=0.0018656049153867003  ParameterDataTypeMode=Specify via dialog  ParameterDataType=float('double')  ParamDataTypeStr=float('double')  OutScaling=1  RndMeth=Nearest  SaturateOnIntegerOverflow=on  OutDataTypeStr=Inherit: Same as input
  b(229) : Gain  Gain=0.0018697485373093468  ParameterDataTypeMode=Specify via dialog  ParameterDataType=float('double')  ParamDataTypeStr=float('double')  OutScaling=1  RndMeth=Nearest  SaturateOnIntegerOverflow=on  OutDataTypeStr=Inherit: Same as input
  b(23) : Gain  Gain=0.0015527270089122293  ParameterDataTypeMode=Specify via dialog  ParameterDataType=float('double')  ParamDataTypeStr=float('double')  OutScaling=1  RndMeth=Nearest  SaturateOnIntegerOverflow=on  OutDataTypeStr=Inherit: Same as input
  b(230) : Gain  Gain=0.0018643076590201808  ParameterDataTypeMode=Specify via dialog  ParameterDataType=float('double')  ParamDataTypeStr=float('double')  OutScaling=1  RndMeth=Nearest  SaturateOnIntegerOverflow=on  OutDataTypeStr=Inherit: Same as input
  b(231) : Gain  Gain=0.0018500595835499061  ParameterDataTypeMode=Specify via dialog  ParameterDataType=float('double')  ParamDataTypeStr=float('double')  OutScaling=1  RndMeth=Nearest  SaturateOnIntegerOverflow=on  OutDataTypeStr=Inherit: Same as input
  b(232) : Gain  Gain=0.001827284713716514  ParameterDataTypeMode=Specify via dialog  ParameterDataType=float('double')  ParamDataTypeStr=float('double')  OutScaling=1  RndMeth=Nearest  SaturateOnIntegerOverflow=on  OutDataTypeStr=Inherit: Same as input
  b(233) : Gain  Gain=0.0017970037296038788  ParameterDataTypeMode=Specify via dialog  ParameterDataType=float('double')  ParamDataTypeStr=float('double')  OutScaling=1  RndMeth=Nearest  SaturateOnIntegerOverflow=on  OutDataTypeStr=Inherit: Same as input
  b(234) : Gain  Gain=0.0017594860519420377  ParameterDataTypeMode=Specify via dialog  ParameterDataType=float('double')  ParamDataTypeStr=float('double')  OutScaling=1  RndMeth=Nearest  SaturateOnIntegerOverflow=on  OutDataTypeStr=Inherit: Same as input
  b(235) : Gain  Gain=0.0017156673234304445  ParameterDataTypeMode=Specify via dialog  ParameterDataType=float('double')  ParamDataTypeStr=float('double')  OutScaling=1  RndMeth=Nearest  SaturateOnIntegerOverflow=on  OutDataTypeStr=Inherit: Same as input
  b(236) : Gain  Gain=0.0016663503114384992  ParameterDataTypeMode=Specify via dialog  ParameterDataType=float('double')  ParamDataTypeStr=float('double')  OutScaling=1  RndMeth=Nearest  SaturateOnIntegerOverflow=on  OutDataTypeStr=Inherit: Same as input
  b(237) : Gain  Gain=0.0016116014194011076  ParameterDataTypeMode=Specify via dialog  ParameterDataType=float('double')  ParamDataTypeStr=float('double')  OutScaling=1  RndMeth=Nearest  SaturateOnIntegerOverflow=on  OutDataTypeStr=Inherit: Same as input
  b(238) : Gain  Gain=0.0015527270089122293  ParameterDataTypeMode=Specify via dialog  ParameterDataType=float('double')  ParamDataTypeStr=float('double')  OutScaling=1  RndMeth=Nearest  SaturateOnIntegerOverflow=on  OutDataTypeStr=Inherit: Same as input
  b(239) : Gain  Gain=0.0014902408540535053  ParameterDataTypeMode=Specify via dialog  ParameterDataType=float('double')  ParamDataTypeStr=float('double')  OutScaling=1  RndMeth=Nearest  SaturateOnIntegerOverflow=on  OutDataTypeStr=Inherit: Same as input
  b(24) : Gain  Gain=0.0016116014194011076  ParameterDataTypeMode=Specify via dialog  ParameterDataType=float('double')  ParamDataTypeStr=float('double')  OutScaling=1  RndMeth=Nearest  SaturateOnIntegerOverflow=on  OutDataTypeStr=Inherit: Same as input
  b(240) : Gain  Gain=0.0014245835558915126  ParameterDataTypeMode=Specify via dialog  ParameterDataType=float('double')  ParamDataTypeStr=float('double')  OutScaling=1  RndMeth=Nearest  SaturateOnIntegerOverflow=on  OutDataTypeStr=Inherit: Same as input
  b(241) : Gain  Gain=0.0013564706827517313  ParameterDataTypeMode=Specify via dialog  ParameterDataType=float('double')  ParamDataTypeStr=float('double')  OutScaling=1  RndMeth=Nearest  SaturateOnIntegerOverflow=on  OutDataTypeStr=Inherit: Same as input
  b(242) : Gain  Gain=0.0012865512850236843  ParameterDataTypeMode=Specify via dialog  ParameterDataType=float('double')  ParamDataTypeStr=float('double')  OutScaling=1  RndMeth=Nearest  SaturateOnIntegerOverflow=on  OutDataTypeStr=Inherit: Same as input
  b(243) : Gain  Gain=0.001215524986978665  ParameterDataTypeMode=Specify via dialog  ParameterDataType=float('double')  ParamDataTypeStr=float('double')  OutScaling=1  RndMeth=Nearest  SaturateOnIntegerOverflow=on  OutDataTypeStr=Inherit: Same as input
  b(244) : Gain  Gain=0.0011435663265835921  ParameterDataTypeMode=Specify via dialog  ParameterDataType=float('double')  ParamDataTypeStr=float('double')  OutScaling=1  RndMeth=Nearest  SaturateOnIntegerOverflow=on  OutDataTypeStr=Inherit: Same as input
  b(245) : Gain  Gain=0.0010715809286023286  ParameterDataTypeMode=Specify via dialog  ParameterDataType=float('double')  ParamDataTypeStr=float('double')  OutScaling=1  RndMeth=Nearest  SaturateOnIntegerOverflow=on  OutDataTypeStr=Inherit: Same as input
  b(246) : Gain  Gain=0.00099957917679242272  ParameterDataTypeMode=Specify via dialog  ParameterDataType=float('double')  ParamDataTypeStr=float('double')  OutScaling=1  RndMeth=Nearest  SaturateOnIntegerOverflow=on  OutDataTypeStr=Inherit: Same as input
  b(247) : Gain  Gain=0.000928205688470267  ParameterDataTypeMode=Specify via dialog  ParameterDataType=float('double')  ParamDataTypeStr=float('double')  OutScaling=1  RndMeth=Nearest  SaturateOnIntegerOverflow=on  OutDataTypeStr=Inherit: Same as input
  b(248) : Gain  Gain=0.00085906126191019659  ParameterDataTypeMode=Specify via dialog  ParameterDataType=float('double')  ParamDataTypeStr=float('double')  OutScaling=1  RndMeth=Nearest  SaturateOnIntegerOverflow=on  OutDataTypeStr=Inherit: Same as input
  b(249) : Gain  Gain=0.00078945898775655888  ParameterDataTypeMode=Specify via dialog  ParameterDataType=float('double')  ParamDataTypeStr=float('double')  OutScaling=1  RndMeth=Nearest  SaturateOnIntegerOverflow=on  OutDataTypeStr=Inherit: Same as input
  b(25) : Gain  Gain=0.0016663503114384992  ParameterDataTypeMode=Specify via dialog  ParameterDataType=float('double')  ParamDataTypeStr=float('double')  OutScaling=1  RndMeth=Nearest  SaturateOnIntegerOverflow=on  OutDataTypeStr=Inherit: Same as input
  b(250) : Gain  Gain=0.00072315700075571872  ParameterDataTypeMode=Specify via dialog  ParameterDataType=float('double')  ParamDataTypeStr=float('double')  OutScaling=1  RndMeth=Nearest  SaturateOnIntegerOverflow=on  OutDataTypeStr=Inherit: Same as input
  b(251) : Gain  Gain=0.00065890295760926093  ParameterDataTypeMode=Specify via dialog  ParameterDataType=float('double')  ParamDataTypeStr=float('double')  OutScaling=1  RndMeth=Nearest  SaturateOnIntegerOverflow=on  OutDataTypeStr=Inherit: Same as input
  b(252) : Gain  Gain=0.00059698927412459089  ParameterDataTypeMode=Specify via dialog  ParameterDataType=float('double')  ParamDataTypeStr=float('double')  OutScaling=1  RndMeth=Nearest  SaturateOnIntegerOverflow=on  OutDataTypeStr=Inherit: Same as input
  b(253) : Gain  Gain=0.0005372270121661929  ParameterDataTypeMode=Specify via dialog  ParameterDataType=float('double')  ParamDataTypeStr=float('double')  OutScaling=1  RndMeth=Nearest  SaturateOnIntegerOverflow=on  OutDataTypeStr=Inherit: Same as input
  b(254) : Gain  Gain=0.00048069537023599302  ParameterDataTypeMode=Specify via dialog  ParameterDataType=float('double')  ParamDataTypeStr=float('double')  OutScaling=1  RndMeth=Nearest  SaturateOnIntegerOverflow=on  OutDataTypeStr=Inherit: Same as input
  b(255) : Gain  Gain=0.00042712643581644722  ParameterDataTypeMode=Specify via dialog  ParameterDataType=float('double')  ParamDataTypeStr=float('double')  OutScaling=1  RndMeth=Nearest  SaturateOnIntegerOverflow=on  OutDataTypeStr=Inherit: Same as input
  b(256) : Gain  Gain=0.00037687532322451843  ParameterDataTypeMode=Specify via dialog  ParameterDataType=float('double')  ParamDataTypeStr=float('double')  OutScaling=1  RndMeth=Nearest  SaturateOnIntegerOverflow=on  OutDataTypeStr=Inherit: Same as input
  b(257) : Gain  Gain=0.00032944657837589384  ParameterDataTypeMode=Specify via dialog  ParameterDataType=float('double')  ParamDataTypeStr=float('double')  OutScaling=1  RndMeth=Nearest  SaturateOnIntegerOverflow=on  OutDataTypeStr=Inherit: Same as input
  b(258) : Gain  Gain=0.00028529534441069443  ParameterDataTypeMode=Specify via dialog  ParameterDataType=float('double')  ParamDataTypeStr=float('double')  OutScaling=1  RndMeth=Nearest  SaturateOnIntegerOverflow=on  OutDataTypeStr=Inherit: Same as input
  b(259) : Gain  Gain=0.00024423156750045524  ParameterDataTypeMode=Specify via dialog  ParameterDataType=float('double')  ParamDataTypeStr=float('double')  OutScaling=1  RndMeth=Nearest  SaturateOnIntegerOverflow=on  OutDataTypeStr=Inherit: Same as input
  b(26) : Gain  Gain=0.0017156673234304445  ParameterDataTypeMode=Specify via dialog  ParameterDataType=float('double')  ParamDataTypeStr=float('double')  OutScaling=1  RndMeth=Nearest  SaturateOnIntegerOverflow=on  OutDataTypeStr=Inherit: Same as input
  b(260) : Gain  Gain=0.00070417510961843762  ParameterDataTypeMode=Specify via dialog  ParameterDataType=float('double')  ParamDataTypeStr=float('double')  OutScaling=1  RndMeth=Nearest  SaturateOnIntegerOverflow=on  OutDataTypeStr=Inherit: Same as input
  b(27) : Gain  Gain=0.0017594860519420377  ParameterDataTypeMode=Specify via dialog  ParameterDataType=float('double')  ParamDataTypeStr=float('double')  OutScaling=1  RndMeth=Nearest  SaturateOnIntegerOverflow=on  OutDataTypeStr=Inherit: Same as input
  b(28) : Gain  Gain=0.0017970037296038788  ParameterDataTypeMode=Specify via dialog  ParameterDataType=float('double')  ParamDataTypeStr=float('double')  OutScaling=1  RndMeth=Nearest  SaturateOnIntegerOverflow=on  OutDataTypeStr=Inherit: Same as input
  b(29) : Gain  Gain=0.001827284713716514  ParameterDataTypeMode=Specify via dialog  ParameterDataType=float('double')  ParamDataTypeStr=float('double')  OutScaling=1  RndMeth=Nearest  SaturateOnIntegerOverflow=on  OutDataTypeStr=Inherit: Same as input
  b(3) : Gain  Gain=0.00028529534441069443  ParameterDataTypeMode=Specify via dialog  ParameterDataType=float('double')  ParamDataTypeStr=float('double')  OutScaling=1  RndMeth=Nearest  SaturateOnIntegerOverflow=on  OutDataTypeStr=Inherit: Same as input
  b(30) : Gain  Gain=0.0018500595835499061  ParameterDataTypeMode=Specify via dialog  ParameterDataType=float('double')  ParamDataTypeStr=float('double')  OutScaling=1  RndMeth=Nearest  SaturateOnIntegerOverflow=on  OutDataTypeStr=Inherit: Same as input
  b(31) : Gain  Gain=0.0018643076590201808  ParameterDataTypeMode=Specify via dialog  ParameterDataType=float('double')  ParamDataTypeStr=float('double')  OutScaling=1  RndMeth=Nearest  SaturateOnIntegerOverflow=on  OutDataTypeStr=Inherit: Same as input
  b(32) : Gain  Gain=0.0018697485373093468  ParameterDataTypeMode=Specify via dialog  ParameterDataType=float('double')  ParamDataTypeStr=float('double')  OutScaling=1  RndMeth=Nearest  SaturateOnIntegerOverflow=on  OutDataTypeStr=Inherit: Same as input
  b(33) : Gain  Gain=0.0018656049153867003  ParameterDataTypeMode=Specify via dialog  ParameterDataType=float('double')  ParamDataTypeStr=float('double')  OutScaling=1  RndMeth=Nearest  SaturateOnIntegerOverflow=on  OutDataTypeStr=Inherit: Same as input
  b(34) : Gain  Gain=0.0018513900016270467  ParameterDataTypeMode=Specify via dialog  ParameterDataType=float('double')  ParamDataTypeStr=float('double')  OutScaling=1  RndMeth=Nearest  SaturateOnIntegerOverflow=on  OutDataTypeStr=Inherit: Same as input
  b(35) : Gain  Gain=0.0018264374579876998  ParameterDataTypeMode=Specify via dialog  ParameterDataType=float('double')  ParamDataTypeStr=float('double')  OutScaling=1  RndMeth=Nearest  SaturateOnIntegerOverflow=on  OutDataTypeStr=Inherit: Same as input
  b(36) : Gain  Gain=0.0017904755880180506  ParameterDataTypeMode=Specify via dialog  ParameterDataType=float('double')  ParamDataTypeStr=float('double')  OutScaling=1  RndMeth=Nearest  SaturateOnIntegerOverflow=on  OutDataTypeStr=Inherit: Same as input
  b(37) : Gain  Gain=0.0017429852808810774  ParameterDataTypeMode=Specify via dialog  ParameterDataType=float('double')  ParamDataTypeStr=float('double')  OutScaling=1  RndMeth=Nearest  SaturateOnIntegerOverflow=on  OutDataTypeStr=Inherit: Same as input
  b(38) : Gain  Gain=0.0016834467566769996  ParameterDataTypeMode=Specify via dialog  ParameterDataType=float('double')  ParamDataTypeStr=float('double')  OutScaling=1  RndMeth=Nearest  SaturateOnIntegerOverflow=on  OutDataTypeStr=Inherit: Same as input
  b(39) : Gain  Gain=0.0016116862849141164  ParameterDataTypeMode=Specify via dialog  ParameterDataType=float('double')  ParamDataTypeStr=float('double')  OutScaling=1  RndMeth=Nearest  SaturateOnIntegerOverflow=on  OutDataTypeStr=Inherit: Same as input
  b(4) : Gain  Gain=0.00032944657837589384  ParameterDataTypeMode=Specify via dialog  ParameterDataType=float('double')  ParamDataTypeStr=float('double')  OutScaling=1  RndMeth=Nearest  SaturateOnIntegerOverflow=on  OutDataTypeStr=Inherit: Same as input
  b(40) : Gain  Gain=0.0015275027261476678  ParameterDataTypeMode=Specify via dialog  ParameterDataType=float('double')  ParamDataTypeStr=float('double')  OutScaling=1  RndMeth=Nearest  SaturateOnIntegerOverflow=on  OutDataTypeStr=Inherit: Same as input
  b(41) : Gain  Gain=0.001430483050405896  ParameterDataTypeMode=Specify via dialog  ParameterDataType=float('double')  ParamDataTypeStr=float('double')  OutScaling=1  RndMeth=Nearest  SaturateOnIntegerOverflow=on  OutDataTypeStr=Inherit: Same as input
  b(42) : Gain  Gain=0.0013208346129694928  ParameterDataTypeMode=Specify via dialog  ParameterDataType=float('double')  ParamDataTypeStr=float('double')  OutScaling=1  RndMeth=Nearest  SaturateOnIntegerOverflow=on  OutDataTypeStr=Inherit: Same as input
  b(43) : Gain  Gain=0.0011982302848979744  ParameterDataTypeMode=Specify via dialog  ParameterDataType=float('double')  ParamDataTypeStr=float('double')  OutScaling=1  RndMeth=Nearest  SaturateOnIntegerOverflow=on  OutDataTypeStr=Inherit: Same as input
  b(44) : Gain  Gain=0.001063020174163772  ParameterDataTypeMode=Specify via dialog  ParameterDataType=float('double')  ParamDataTypeStr=float('double')  OutScaling=1  RndMeth=Nearest  SaturateOnIntegerOverflow=on  OutDataTypeStr=Inherit: Same as input
  b(45) : Gain  Gain=0.00091520468672270927  ParameterDataTypeMode=Specify via dialog  ParameterDataType=float('double')  ParamDataTypeStr=float('double')  OutScaling=1  RndMeth=Nearest  SaturateOnIntegerOverflow=on  OutDataTypeStr=Inherit: Same as input
  b(46) : Gain  Gain=0.00075512721901295162  ParameterDataTypeMode=Specify via dialog  ParameterDataType=float('double')  ParamDataTypeStr=float('double')  OutScaling=1  RndMeth=Nearest  SaturateOnIntegerOverflow=on  OutDataTypeStr=Inherit: Same as input
  b(47) : Gain  Gain=0.00058302352831076721  ParameterDataTypeMode=Specify via dialog  ParameterDataType=float('double')  ParamDataTypeStr=float('double')  OutScaling=1  RndMeth=Nearest  SaturateOnIntegerOverflow=on  OutDataTypeStr=Inherit: Same as input
  b(48) : Gain  Gain=0.00039951833019874391  ParameterDataTypeMode=Specify via dialog  ParameterDataType=float('double')  ParamDataTypeStr=float('double')  OutScaling=1  RndMeth=Nearest  SaturateOnIntegerOverflow=on  OutDataTypeStr=Inherit: Same as input
  b(49) : Gain  Gain=0.00020504503595217299  ParameterDataTypeMode=Specify via dialog  ParameterDataType=float('double')  ParamDataTypeStr=float('double')  OutScaling=1  RndMeth=Nearest  SaturateOnIntegerOverflow=on  OutDataTypeStr=Inherit: Same as input
  b(5) : Gain  Gain=0.00037687532322451843  ParameterDataTypeMode=Specify via dialog  ParameterDataType=float('double')  ParamDataTypeStr=float('double')  OutScaling=1  RndMeth=Nearest  SaturateOnIntegerOverflow=on  OutDataTypeStr=Inherit: Same as input
  b(50) : Gain  Gain=2.4895367239561282e-007  ParameterDataTypeMode=Specify via dialog  ParameterDataType=float('double')  ParamDataTypeStr=float('double')  OutScaling=1  RndMeth=Nearest  SaturateOnIntegerOverflow=on  OutDataTypeStr=Inherit: Same as input
  b(51) : Gain  Gain=-0.00021409722155803576  ParameterDataTypeMode=Specify via dialog  ParameterDataType=float('double')  ParamDataTypeStr=float('double')  OutScaling=1  RndMeth=Nearest  SaturateOnIntegerOverflow=on  OutDataTypeStr=Inherit: Same as input
  b(52) : Gain  Gain=-0.00043706573064342683  ParameterDataTypeMode=Specify via dialog  ParameterDataType=float('double')  ParamDataTypeStr=float('double')  OutScaling=1  RndMeth=Nearest  SaturateOnIntegerOverflow=on  OutDataTypeStr=Inherit: Same as input
  b(53) : Gain  Gain=-0.00066787760762591962  ParameterDataTypeMode=Specify via dialog  ParameterDataType=float('double')  ParamDataTypeStr=float('double')  OutScaling=1  RndMeth=Nearest  SaturateOnIntegerOverflow=on  OutDataTypeStr=Inherit: Same as input
  b(54) : Gain  Gain=-0.0009052529655871384  ParameterDataTypeMode=Specify via dialog  ParameterDataType=float('double')  ParamDataTypeStr=float('double')  OutScaling=1  RndMeth=Nearest  SaturateOnIntegerOverflow=on  OutDataTypeStr=Inherit: Same as input
  b(55) : Gain  Gain=-0.0011482695116857549  ParameterDataTypeMode=Specify via dialog  ParameterDataType=float('double')  ParamDataTypeStr=float('double')  OutScaling=1  RndMeth=Nearest  SaturateOnIntegerOverflow=on  OutDataTypeStr=Inherit: Same as input
  b(56) : Gain  Gain=-0.0013954701655563839  ParameterDataTypeMode=Specify via dialog  ParameterDataType=float('double')  ParamDataTypeStr=float('double')  OutScaling=1  RndMeth=Nearest  SaturateOnIntegerOverflow=on  OutDataTypeStr=Inherit: Same as input
  b(57) : Gain  Gain=-0.0016456276040868589  ParameterDataTypeMode=Specify via dialog  ParameterDataType=float('double')  ParamDataTypeStr=float('double')  OutScaling=1  RndMeth=Nearest  SaturateOnIntegerOverflow=on  OutDataTypeStr=Inherit: Same as input
  b(58) : Gain  Gain=-0.0018972524976453848  ParameterDataTypeMode=Specify via dialog  ParameterDataType=float('double')  ParamDataTypeStr=float('double')  OutScaling=1  RndMeth=Nearest  SaturateOnIntegerOverflow=on  OutDataTypeStr=Inherit: Same as input
  b(59) : Gain  Gain=-0.002148902815176169  ParameterDataTypeMode=Specify via dialog  ParameterDataType=float('double')  ParamDataTypeStr=float('double')  OutScaling=1  RndMeth=Nearest  SaturateOnIntegerOverflow=on  OutDataTypeStr=Inherit: Same as input
  b(6) : Gain  Gain=0.00042712643581644722  ParameterDataTypeMode=Specify via dialog  ParameterDataType=float('double')  ParamDataTypeStr=float('double')  OutScaling=1  RndMeth=Nearest  SaturateOnIntegerOverflow=on  OutDataTypeStr=Inherit: Same as input
  b(60) : Gain  Gain=-0.0023988698157260263  ParameterDataTypeMode=Specify via dialog  ParameterDataType=float('double')  ParamDataTypeStr=float('double')  OutScaling=1  RndMeth=Nearest  SaturateOnIntegerOverflow=on  OutDataTypeStr=Inherit: Same as input
  b(61) : Gain  Gain=-0.0026455884436352908  ParameterDataTypeMode=Specify via dialog  ParameterDataType=float('double')  ParamDataTypeStr=float('double')  OutScaling=1  RndMeth=Nearest  SaturateOnIntegerOverflow=on  OutDataTypeStr=Inherit: Same as input
  b(62) : Gain  Gain=-0.0028873200222469617  ParameterDataTypeMode=Specify via dialog  ParameterDataType=float('double')  ParamDataTypeStr=float('double')  OutScaling=1  RndMeth=Nearest  SaturateOnIntegerOverflow=on  OutDataTypeStr=Inherit: Same as input
  b(63) : Gain  Gain=-0.0031222962030929349  ParameterDataTypeMode=Specify via dialog  ParameterDataType=float('double')  ParamDataTypeStr=float('double')  OutScaling=1  RndMeth=Nearest  SaturateOnIntegerOverflow=on  OutDataTypeStr=Inherit: Same as input
  b(64) : Gain  Gain=-0.0033486524967329487  ParameterDataTypeMode=Specify via dialog  ParameterDataType=float('double')  ParamDataTypeStr=float('double')  OutScaling=1  RndMeth=Nearest  SaturateOnIntegerOverflow=on  OutDataTypeStr=Inherit: Same as input
  b(65) : Gain  Gain=-0.0035646528383071309  ParameterDataTypeMode=Specify via dialog  ParameterDataType=float('double')  ParamDataTypeStr=float('double')  OutScaling=1  RndMeth=Nearest  SaturateOnIntegerOverflow=on  OutDataTypeStr=Inherit: Same as input
  b(66) : Gain  Gain=-0.0037682781895092285  ParameterDataTypeMode=Specify via dialog  ParameterDataType=float('double')  ParamDataTypeStr=float('double')  OutScaling=1  RndMeth=Nearest  SaturateOnIntegerOverflow=on  OutDataTypeStr=Inherit: Same as input
  b(67) : Gain  Gain=-0.0039577961713118419  ParameterDataTypeMode=Specify via dialog  ParameterDataType=float('double')  ParamDataTypeStr=float('double')  OutScaling=1  RndMeth=Nearest  SaturateOnIntegerOverflow=on  OutDataTypeStr=Inherit: Same as input
  b(68) : Gain  Gain=-0.0041311777625552227  ParameterDataTypeMode=Specify via dialog  ParameterDataType=float('double')  ParamDataTypeStr=float('double')  OutScaling=1  RndMeth=Nearest  SaturateOnIntegerOverflow=on  OutDataTypeStr=Inherit: Same as input
  b(69) : Gain  Gain=-0.0042865991428804734  ParameterDataTypeMode=Specify via dialog  ParameterDataType=float('double')  ParamDataTypeStr=float('double')  OutScaling=1  RndMeth=Nearest  SaturateOnIntegerOverflow=on  OutDataTypeStr=Inherit: Same as input
  b(7) : Gain  Gain=0.00048069537023599302  ParameterDataTypeMode=Specify via dialog  ParameterDataType=float('double')  ParamDataTypeStr=float('double')  OutScaling=1  RndMeth=Nearest  SaturateOnIntegerOverflow=on  OutDataTypeStr=Inherit: Same as input
  b(70) : Gain  Gain=-0.0044221700763802108  ParameterDataTypeMode=Specify via dialog  ParameterDataType=float('double')  ParamDataTypeStr=float('double')  OutScaling=1  RndMeth=Nearest  SaturateOnIntegerOverflow=on  OutDataTypeStr=Inherit: Same as input
  b(71) : Gain  Gain=-0.004536068879832213  ParameterDataTypeMode=Specify via dialog  ParameterDataType=float('double')  ParamDataTypeStr=float('double')  OutScaling=1  RndMeth=Nearest  SaturateOnIntegerOverflow=on  OutDataTypeStr=Inherit: Same as input
  b(72) : Gain  Gain=-0.0046264252289973861  ParameterDataTypeMode=Specify via dialog  ParameterDataType=float('double')  ParamDataTypeStr=float('double')  OutScaling=1  RndMeth=Nearest  SaturateOnIntegerOverflow=on  OutDataTypeStr=Inherit: Same as input
  b(73) : Gain  Gain=-0.0046915387161280356  ParameterDataTypeMode=Specify via dialog  ParameterDataType=float('double')  ParamDataTypeStr=float('double')  OutScaling=1  RndMeth=Nearest  SaturateOnIntegerOverflow=on  OutDataTypeStr=Inherit: Same as input
  b(74) : Gain  Gain=-0.0047297082884658788  ParameterDataTypeMode=Specify via dialog  ParameterDataType=float('double')  ParamDataTypeStr=float('double')  OutScaling=1  RndMeth=Nearest  SaturateOnIntegerOverflow=on  OutDataTypeStr=Inherit: Same as input
  b(75) : Gain  Gain=-0.0047393103130561991  ParameterDataTypeMode=Specify via dialog  ParameterDataType=float('double')  ParamDataTypeStr=float('double')  OutScaling=1  RndMeth=Nearest  SaturateOnIntegerOverflow=on  OutDataTypeStr=Inherit: Same as input
  b(76) : Gain  Gain=-0.0047188020939299127  ParameterDataTypeMode=Specify via dialog  ParameterDataType=float('double')  ParamDataTypeStr=float('double')  OutScaling=1  RndMeth=Nearest  SaturateOnIntegerOverflow=on  OutDataTypeStr=Inherit: Same as input
  b(77) : Gain  Gain=-0.0046668113226438135  ParameterDataTypeMode=Specify via dialog  ParameterDataType=float('double')  ParamDataTypeStr=float('double')  OutScaling=1  RndMeth=Nearest  SaturateOnIntegerOverflow=on  OutDataTypeStr=Inherit: Same as input
  b(78) : Gain  Gain=-0.0045819428812625337  ParameterDataTypeMode=Specify via dialog  ParameterDataType=float('double')  ParamDataTypeStr=float('double')  OutScaling=1  RndMeth=Nearest  SaturateOnIntegerOverflow=on  OutDataTypeStr=Inherit: Same as input
  b(79) : Gain  Gain=-0.0044630950959934825  ParameterDataTypeMode=Specify via dialog  ParameterDataType=float('double')  ParamDataTypeStr=float('double')  OutScaling=1  RndMeth=Nearest  SaturateOnIntegerOverflow=on  OutDataTypeStr=Inherit: Same as input
  b(8) : Gain  Gain=0.0005372270121661929  ParameterDataTypeMode=Specify via dialog  ParameterDataType=float('double')  ParamDataTypeStr=float('double')  OutScaling=1  RndMeth=Nearest  SaturateOnIntegerOverflow=on  OutDataTypeStr=Inherit: Same as input
  b(80) : Gain  Gain=-0.0043091320843662781  ParameterDataTypeMode=Specify via dialog  ParameterDataType=float('double')  ParamDataTypeStr=float('double')  OutScaling=1  RndMeth=Nearest  SaturateOnIntegerOverflow=on  OutDataTypeStr=Inherit: Same as input
  b(81) : Gain  Gain=-0.0041191558942448771  ParameterDataTypeMode=Specify via dialog  ParameterDataType=float('double')  ParamDataTypeStr=float('double')  OutScaling=1  RndMeth=Nearest  SaturateOnIntegerOverflow=on  OutDataTypeStr=Inherit: Same as input
  b(82) : Gain  Gain=-0.0038924172738207274  ParameterDataTypeMode=Specify via dialog  ParameterDataType=float('double')  ParamDataTypeStr=float('double')  OutScaling=1  RndMeth=Nearest  SaturateOnIntegerOverflow=on  OutDataTypeStr=Inherit: Same as input
  b(83) : Gain  Gain=-0.0036282918249470573  ParameterDataTypeMode=Specify via dialog  ParameterDataType=float('double')  ParamDataTypeStr=float('double')  OutScaling=1  RndMeth=Nearest  SaturateOnIntegerOverflow=on  OutDataTypeStr=Inherit: Same as input
  b(84) : Gain  Gain=-0.0033263178221817377  ParameterDataTypeMode=Specify via dialog  ParameterDataType=float('double')  ParamDataTypeStr=float('double')  OutScaling=1  RndMeth=Nearest  SaturateOnIntegerOverflow=on  OutDataTypeStr=Inherit: Same as input
  b(85) : Gain  Gain=-0.0029862469165041388  ParameterDataTypeMode=Specify via dialog  ParameterDataType=float('double')  ParamDataTypeStr=float('double')  OutScaling=1  RndMeth=Nearest  SaturateOnIntegerOverflow=on  OutDataTypeStr=Inherit: Same as input
  b(86) : Gain  Gain=-0.0026079964847781222  ParameterDataTypeMode=Specify via dialog  ParameterDataType=float('double')  ParamDataTypeStr=float('double')  OutScaling=1  RndMeth=Nearest  SaturateOnIntegerOverflow=on  OutDataTypeStr=Inherit: Same as input
  b(87) : Gain  Gain=-0.0021916374965953132  ParameterDataTypeMode=Specify via dialog  ParameterDataType=float('double')  ParamDataTypeStr=float('double')  OutScaling=1  RndMeth=Nearest  SaturateOnIntegerOverflow=on  OutDataTypeStr=Inherit: Same as input
  b(88) : Gain  Gain=-0.0017374680097337761  ParameterDataTypeMode=Specify via dialog  ParameterDataType=float('double')  ParamDataTypeStr=float('double')  OutScaling=1  RndMeth=Nearest  SaturateOnIntegerOverflow=on  OutDataTypeStr=Inherit: Same as input
  b(89) : Gain  Gain=-0.0012459755928315391  ParameterDataTypeMode=Specify via dialog  ParameterDataType=float('double')  ParamDataTypeStr=float('double')  OutScaling=1  RndMeth=Nearest  SaturateOnIntegerOverflow=on  OutDataTypeStr=Inherit: Same as input
  b(9) : Gain  Gain=0.00059698927412459089  ParameterDataTypeMode=Specify via dialog  ParameterDataType=float('double')  ParamDataTypeStr=float('double')  OutScaling=1  RndMeth=Nearest  SaturateOnIntegerOverflow=on  OutDataTypeStr=Inherit: Same as input
  b(90) : Gain  Gain=-0.00071779930929411525  ParameterDataTypeMode=Specify via dialog  ParameterDataType=float('double')  ParamDataTypeStr=float('double')  OutScaling=1  RndMeth=Nearest  SaturateOnIntegerOverflow=on  OutDataTypeStr=Inherit: Same as input
  b(91) : Gain  Gain=-0.00015384920636331843  ParameterDataTypeMode=Specify via dialog  ParameterDataType=float('double')  ParamDataTypeStr=float('double')  OutScaling=1  RndMeth=Nearest  SaturateOnIntegerOverflow=on  OutDataTypeStr=Inherit: Same as input
  b(92) : Gain  Gain=0.00044484680086729451  ParameterDataTypeMode=Specify via dialog  ParameterDataType=float('double')  ParamDataTypeStr=float('double')  OutScaling=1  RndMeth=Nearest  SaturateOnIntegerOverflow=on  OutDataTypeStr=Inherit: Same as input
  b(93) : Gain  Gain=0.0010770433381879106  ParameterDataTypeMode=Specify via dialog  ParameterDataType=float('double')  ParamDataTypeStr=float('double')  OutScaling=1  RndMeth=Nearest  SaturateOnIntegerOverflow=on  OutDataTypeStr=Inherit: Same as input
  b(94) : Gain  Gain=0.0017412535010850488  ParameterDataTypeMode=Specify via dialog  ParameterDataType=float('double')  ParamDataTypeStr=float('double')  OutScaling=1  RndMeth=Nearest  SaturateOnIntegerOverflow=on  OutDataTypeStr=Inherit: Same as input
  b(95) : Gain  Gain=0.0024358839160543953  ParameterDataTypeMode=Specify via dialog  ParameterDataType=float('double')  ParamDataTypeStr=float('double')  OutScaling=1  RndMeth=Nearest  SaturateOnIntegerOverflow=on  OutDataTypeStr=Inherit: Same as input
  b(96) : Gain  Gain=0.0031591101868804696  ParameterDataTypeMode=Specify via dialog  ParameterDataType=float('double')  ParamDataTypeStr=float('double')  OutScaling=1  RndMeth=Nearest  SaturateOnIntegerOverflow=on  OutDataTypeStr=Inherit: Same as input
  b(97) : Gain  Gain=0.003908939056141314  ParameterDataTypeMode=Specify via dialog  ParameterDataType=float('double')  ParamDataTypeStr=float('double')  OutScaling=1  RndMeth=Nearest  SaturateOnIntegerOverflow=on  OutDataTypeStr=Inherit: Same as input
  b(98) : Gain  Gain=0.0046831909839310645  ParameterDataTypeMode=Specify via dialog  ParameterDataType=float('double')  ParamDataTypeStr=float('double')  OutScaling=1  RndMeth=Nearest  SaturateOnIntegerOverflow=on  OutDataTypeStr=Inherit: Same as input
  b(99) : Gain  Gain=0.0054795719185856736  ParameterDataTypeMode=Specify via dialog  ParameterDataType=float('double')  ParamDataTypeStr=float('double')  OutScaling=1  RndMeth=Nearest  SaturateOnIntegerOverflow=on  OutDataTypeStr=Inherit: Same as input
  Output : Outport
  wires:
  Input/1 -> b(1)/1, BodyDelay2/1
  b(1)/1 -> BodyLSum2/2
  BodyDelay2/1 -> b(2)/1, BodyDelay3/1
  b(2)/1 -> BodyLSum2/1
  BodyLSum2/1 -> BodyLSum3/2
  BodyDelay3/1 -> b(3)/1, BodyDelay4/1
  b(3)/1 -> BodyLSum3/1
  BodyLSum3/1 -> BodyLSum4/2
  BodyDelay4/1 -> b(4)/1, BodyDelay5/1
  b(4)/1 -> BodyLSum4/1
  BodyLSum4/1 -> BodyLSum5/2
  BodyDelay5/1 -> b(5)/1, BodyDelay6/1
  b(5)/1 -> BodyLSum5/1
  BodyLSum5/1 -> BodyLSum6/2
  BodyDelay6/1 -> b(6)/1, BodyDelay7/1
  b(6)/1 -> BodyLSum6/1
  BodyLSum6/1 -> BodyLSum7/2
  BodyDelay7/1 -> b(7)/1, BodyDelay8/1
  b(7)/1 -> BodyLSum7/1
  BodyLSum7/1 -> BodyLSum8/2
  BodyDelay8/1 -> b(8)/1, BodyDelay9/1
  b(8)/1 -> BodyLSum8/1
  BodyLSum8/1 -> BodyLSum9/2
  BodyDelay9/1 -> b(9)/1, BodyDelay10/1
  b(9)/1 -> BodyLSum9/1
  BodyLSum9/1 -> BodyLSum10/2
  BodyDelay10/1 -> b(10)/1, BodyDelay11/1
  b(10)/1 -> BodyLSum10/1
  BodyLSum10/1 -> BodyLSum11/2
  BodyDelay11/1 -> b(11)/1, BodyDelay12/1
  b(11)/1 -> BodyLSum11/1
  BodyLSum11/1 -> BodyLSum12/2
  BodyDelay12/1 -> b(12)/1, BodyDelay13/1
  b(12)/1 -> BodyLSum12/1
  BodyLSum12/1 -> BodyLSum13/2
  BodyDelay13/1 -> b(13)/1, BodyDelay14/1
  b(13)/1 -> BodyLSum13/1
  BodyLSum13/1 -> BodyLSum14/2
  BodyDelay14/1 -> b(14)/1, BodyDelay15/1
  b(14)/1 -> BodyLSum14/1
  BodyLSum14/1 -> BodyLSum15/2
  BodyDelay15/1 -> b(15)/1, BodyDelay16/1
  b(15)/1 -> BodyLSum15/1
  BodyLSum15/1 -> BodyLSum16/2
  BodyDelay16/1 -> b(16)/1, BodyDelay17/1
  b(16)/1 -> BodyLSum16/1
  BodyLSum16/1 -> BodyLSum17/2
  BodyDelay17/1 -> b(17)/1, BodyDelay18/1
  b(17)/1 -> BodyLSum17/1
  BodyLSum17/1 -> BodyLSum18/2
  BodyDelay18/1 -> b(18)/1, BodyDelay19/1
  b(18)/1 -> BodyLSum18/1
  BodyLSum18/1 -> BodyLSum19/2
  BodyDelay19/1 -> b(19)/1, BodyDelay20/1
  b(19)/1 -> BodyLSum19/1
  BodyLSum19/1 -> BodyLSum20/2
  BodyDelay20/1 -> b(20)/1, BodyDelay21/1
  b(20)/1 -> BodyLSum20/1
  BodyLSum20/1 -> BodyLSum21/2
  BodyDelay21/1 -> b(21)/1, BodyDelay22/1
  b(21)/1 -> BodyLSum21/1
  BodyLSum21/1 -> BodyLSum22/2
  BodyDelay22/1 -> b(22)/1, BodyDelay23/1
  b(22)/1 -> BodyLSum22/1
  BodyLSum22/1 -> BodyLSum23/2
  BodyDelay23/1 -> b(23)/1, BodyDelay24/1
  b(23)/1 -> BodyLSum23/1
  BodyLSum23/1 -> BodyLSum24/2
  BodyDelay24/1 -> b(24)/1, BodyDelay25/1
  b(24)/1 -> BodyLSum24/1
  BodyLSum24/1 -> BodyLSum25/2
  BodyDelay25/1 -> b(25)/1, BodyDelay26/1
  b(25)/1 -> BodyLSum25/1
  BodyLSum25/1 -> BodyLSum26/2
  BodyDelay26/1 -> b(26)/1, BodyDelay27/1
  b(26)/1 -> BodyLSum26/1
  BodyLSum26/1 -> BodyLSum27/2
  BodyDelay27/1 -> b(27)/1, BodyDelay28/1
  b(27)/1 -> BodyLSum27/1
  BodyLSum27/1 -> BodyLSum28/2
  BodyDelay28/1 -> b(28)/1, BodyDelay29/1
  b(28)/1 -> BodyLSum28/1
  BodyLSum28/1 -> BodyLSum29/2
  BodyDelay29/1 -> b(29)/1, BodyDelay30/1
  b(29)/1 -> BodyLSum29/1
  BodyLSum29/1 -> BodyLSum30/2
  BodyDelay30/1 -> b(30)/1, BodyDelay31/1
  b(30)/1 -> BodyLSum30/1
  BodyLSum30/1 -> BodyLSum31/2
  BodyDelay31/1 -> b(31)/1, BodyDelay32/1
  b(31)/1 -> BodyLSum31/1
  BodyLSum31/1 -> BodyLSum32/2
  BodyDelay32/1 -> b(32)/1, BodyDelay33/1
  b(32)/1 -> BodyLSum32/1
  BodyLSum32/1 -> BodyLSum33/2
  BodyDelay33/1 -> b(33)/1, BodyDelay34/1
  b(33)/1 -> BodyLSum33/1
  BodyLSum33/1 -> BodyLSum34/2
  BodyDelay34/1 -> b(34)/1, BodyDelay35/1
  b(34)/1 -> BodyLSum34/1
  BodyLSum34/1 -> BodyLSum35/2
  BodyDelay35/1 -> b(35)/1, BodyDelay36/1
  b(35)/1 -> BodyLSum35/1
  BodyLSum35/1 -> BodyLSum36/2
  BodyDelay36/1 -> b(36)/1, BodyDelay37/1
  b(36)/1 -> BodyLSum36/1
  BodyLSum36/1 -> BodyLSum37/2
  BodyDelay37/1 -> b(37)/1, BodyDelay38/1
  b(37)/1 -> BodyLSum37/1
  BodyLSum37/1 -> BodyLSum38/2
  BodyDelay38/1 -> b(38)/1, BodyDelay39/1
  b(38)/1 -> BodyLSum38/1
  BodyLSum38/1 -> BodyLSum39/2
  BodyDelay39/1 -> b(39)/1, BodyDelay40/1
  b(39)/1 -> BodyLSum39/1
  BodyLSum39/1 -> BodyLSum40/2
  BodyDelay40/1 -> b(40)/1, BodyDelay41/1
  b(40)/1 -> BodyLSum40/1
  BodyLSum40/1 -> BodyLSum41/2
  BodyDelay41/1 -> b(41)/1, BodyDelay42/1
  b(41)/1 -> BodyLSum41/1
  BodyLSum41/1 -> BodyLSum42/2
  BodyDelay42/1 -> b(42)/1, BodyDelay43/1
  b(42)/1 -> BodyLSum42/1
  BodyLSum42/1 -> BodyLSum43/2
  BodyDelay43/1 -> b(43)/1, BodyDelay44/1
  b(43)/1 -> BodyLSum43/1
  BodyLSum43/1 -> BodyLSum44/2
  BodyDelay44/1 -> b(44)/1, BodyDelay45/1
  b(44)/1 -> BodyLSum44/1
  BodyLSum44/1 -> BodyLSum45/2
  BodyDelay45/1 -> b(45)/1, BodyDelay46/1
  b(45)/1 -> BodyLSum45/1
  BodyLSum45/1 -> BodyLSum46/2
  BodyDelay46/1 -> b(46)/1, BodyDelay47/1
  b(46)/1 -> BodyLSum46/1
  BodyLSum46/1 -> BodyLSum47/2
  BodyDelay47/1 -> b(47)/1, BodyDelay48/1
  b(47)/1 -> BodyLSum47/1
  BodyLSum47/1 -> BodyLSum48/2
  BodyDelay48/1 -> b(48)/1, BodyDelay49/1
  b(48)/1 -> BodyLSum48/1
  BodyLSum48/1 -> BodyLSum49/2
  BodyDelay49/1 -> b(49)/1, BodyDelay50/1
  b(49)/1 -> BodyLSum49/1
  BodyLSum49/1 -> BodyLSum50/2
  BodyDelay50/1 -> b(50)/1, BodyDelay51/1
  b(50)/1 -> BodyLSum50/1
  BodyLSum50/1 -> BodyLSum51/2
  BodyDelay51/1 -> b(51)/1, BodyDelay52/1
  b(51)/1 -> BodyLSum51/1
  BodyLSum51/1 -> BodyLSum52/2
  BodyDelay52/1 -> b(52)/1, BodyDelay53/1
  b(52)/1 -> BodyLSum52/1
  BodyLSum52/1 -> BodyLSum53/2
  BodyDelay53/1 -> b(53)/1, BodyDelay54/1
  b(53)/1 -> BodyLSum53/1
  BodyLSum53/1 -> BodyLSum54/2
  BodyDelay54/1 -> b(54)/1, BodyDelay55/1
  b(54)/1 -> BodyLSum54/1
  BodyLSum54/1 -> BodyLSum55/2
  BodyDelay55/1 -> b(55)/1, BodyDelay56/1
  b(55)/1 -> BodyLSum55/1
  BodyLSum55/1 -> BodyLSum56/2
  BodyDelay56/1 -> b(56)/1, BodyDelay57/1
  b(56)/1 -> BodyLSum56/1
  BodyLSum56/1 -> BodyLSum57/2
  BodyDelay57/1 -> b(57)/1, BodyDelay58/1
  b(57)/1 -> BodyLSum57/1
  BodyLSum57/1 -> BodyLSum58/2
  BodyDelay58/1 -> b(58)/1, BodyDelay59/1
  b(58)/1 -> BodyLSum58/1
  BodyLSum58/1 -> BodyLSum59/2
  BodyDelay59/1 -> b(59)/1, BodyDelay60/1
  b(59)/1 -> BodyLSum59/1
  BodyLSum59/1 -> BodyLSum60/2
  BodyDelay60/1 -> b(60)/1, BodyDelay61/1
  b(60)/1 -> BodyLSum60/1
  BodyLSum60/1 -> BodyLSum61/2
  BodyDelay61/1 -> b(61)/1, BodyDelay62/1
  b(61)/1 -> BodyLSum61/1
  BodyLSum61/1 -> BodyLSum62/2
  BodyDelay62/1 -> b(62)/1, BodyDelay63/1
  b(62)/1 -> BodyLSum62/1
  BodyLSum62/1 -> BodyLSum63/2
  BodyDelay63/1 -> b(63)/1, BodyDelay64/1
  b(63)/1 -> BodyLSum63/1
  BodyLSum63/1 -> BodyLSum64/2
  BodyDelay64/1 -> b(64)/1, BodyDelay65/1
  b(64)/1 -> BodyLSum64/1
  BodyLSum64/1 -> BodyLSum65/2
  BodyDelay65/1 -> b(65)/1, BodyDelay66/1
  b(65)/1 -> BodyLSum65/1
  BodyLSum65/1 -> BodyLSum66/2
  BodyDelay66/1 -> b(66)/1, BodyDelay67/1
  b(66)/1 -> BodyLSum66/1
  BodyLSum66/1 -> BodyLSum67/2
  BodyDelay67/1 -> b(67)/1, BodyDelay68/1
  b(67)/1 -> BodyLSum67/1
  BodyLSum67/1 -> BodyLSum68/2
  BodyDelay68/1 -> b(68)/1, BodyDelay69/1
  b(68)/1 -> BodyLSum68/1
  BodyLSum68/1 -> BodyLSum69/2
  BodyDelay69/1 -> b(69)/1, BodyDelay70/1
  b(69)/1 -> BodyLSum69/1
  BodyLSum69/1 -> BodyLSum70/2
  BodyDelay70/1 -> b(70)/1, BodyDelay71/1
  b(70)/1 -> BodyLSum70/1
  BodyLSum70/1 -> BodyLSum71/2
  BodyDelay71/1 -> b(71)/1, BodyDelay72/1
  b(71)/1 -> BodyLSum71/1
  BodyLSum71/1 -> BodyLSum72/2
  BodyDelay72/1 -> b(72)/1, BodyDelay73/1
  b(72)/1 -> BodyLSum72/1
  BodyLSum72/1 -> BodyLSum73/2
  BodyDelay73/1 -> b(73)/1, BodyDelay74/1
  b(73)/1 -> BodyLSum73/1
  BodyLSum73/1 -> BodyLSum74/2
  BodyDelay74/1 -> b(74)/1, BodyDelay75/1
  b(74)/1 -> BodyLSum74/1
  BodyLSum74/1 -> BodyLSum75/2
  BodyDelay75/1 -> b(75)/1, BodyDelay76/1
  b(75)/1 -> BodyLSum75/1
  BodyLSum75/1 -> BodyLSum76/2
  BodyDelay76/1 -> b(76)/1, BodyDelay77/1
  b(76)/1 -> BodyLSum76/1
  BodyLSum76/1 -> BodyLSum77/2
  BodyDelay77/1 -> b(77)/1, BodyDelay78/1
  b(77)/1 -> BodyLSum77/1
  BodyLSum77/1 -> BodyLSum78/2
  BodyDelay78/1 -> b(78)/1, BodyDelay79/1
  b(78)/1 -> BodyLSum78/1
  BodyLSum78/1 -> BodyLSum79/2
  BodyDelay79/1 -> b(79)/1, BodyDelay80/1
  b(79)/1 -> BodyLSum79/1
  BodyLSum79/1 -> BodyLSum80/2
  BodyDelay80/1 -> b(80)/1, BodyDelay81/1
  b(80)/1 -> BodyLSum80/1
  BodyLSum80/1 -> BodyLSum81/2
  BodyDelay81/1 -> b(81)/1, BodyDelay82/1
  b(81)/1 -> BodyLSum81/1
  BodyLSum81/1 -> BodyLSum82/2
  BodyDelay82/1 -> b(82)/1, BodyDelay83/1
  b(82)/1 -> BodyLSum82/1
  BodyLSum82/1 -> BodyLSum83/2
  BodyDelay83/1 -> b(83)/1, BodyDelay84/1
  b(83)/1 -> BodyLSum83/1
  BodyLSum83/1 -> BodyLSum84/2
  BodyDelay84/1 -> b(84)/1, BodyDelay85/1
  b(84)/1 -> BodyLSum84/1
  BodyLSum84/1 -> BodyLSum85/2
  BodyDelay85/1 -> b(85)/1, BodyDelay86/1
  b(85)/1 -> BodyLSum85/1
  BodyLSum85/1 -> BodyLSum86/2
  BodyDelay86/1 -> b(86)/1, BodyDelay87/1
  b(86)/1 -> BodyLSum86/1
  BodyLSum86/1 -> BodyLSum87/2
  BodyDelay87/1 -> b(87)/1, BodyDelay88/1
  b(87)/1 -> BodyLSum87/1
  BodyLSum87/1 -> BodyLSum88/2
  BodyDelay88/1 -> b(88)/1, BodyDelay89/1
  b(88)/1 -> BodyLSum88/1
  BodyLSum88/1 -> BodyLSum89/2
  BodyDelay89/1 -> b(89)/1, BodyDelay90/1
  b(89)/1 -> BodyLSum89/1
  BodyLSum89/1 -> BodyLSum90/2
  BodyDelay90/1 -> b(90)/1, BodyDelay91/1
  b(90)/1 -> BodyLSum90/1
  BodyLSum90/1 -> BodyLSum91/2
  BodyDelay91/1 -> b(91)/1, BodyDelay92/1
  b(91)/1 -> BodyLSum91/1
  BodyLSum91/1 -> BodyLSum92/2
  BodyDelay92/1 -> b(92)/1, BodyDelay93/1
  b(92)/1 -> BodyLSum92/1
  BodyLSum92/1 -> BodyLSum93/2
  BodyDelay93/1 -> b(93)/1, BodyDelay94/1
  b(93)/1 -> BodyLSum93/1
  BodyLSum93/1 -> BodyLSum94/2
  BodyDelay94/1 -> b(94)/1, BodyDelay95/1
  b(94)/1 -> BodyLSum94/1
  BodyLSum94/1 -> BodyLSum95/2
  BodyDelay95/1 -> b(95)/1, BodyDelay96/1
  b(95)/1 -> BodyLSum95/1
  BodyLSum95/1 -> BodyLSum96/2
  BodyDelay96/1 -> b(96)/1, BodyDelay97/1
  b(96)/1 -> BodyLSum96/1
  BodyLSum96/1 -> BodyLSum97/2
  BodyDelay97/1 -> b(97)/1, BodyDelay98/1
  b(97)/1 -> BodyLSum97/1
  BodyLSum97/1 -> BodyLSum98/2
  BodyDelay98/1 -> b(98)/1, BodyDelay99/1
  b(98)/1 -> BodyLSum98/1
  BodyLSum98/1 -> BodyLSum99/2
  BodyDelay99/1 -> b(99)/1, BodyDelay100/1
  b(99)/1 -> BodyLSum99/1
  BodyLSum99/1 -> BodyLSum100/2
  BodyDelay100/1 -> b(100)/1, BodyDelay101/1
  b(100)/1 -> BodyLSum100/1
  BodyLSum100/1 -> BodyLSum101/2
  BodyDelay101/1 -> b(101)/1, BodyDelay102/1
  b(101)/1 -> BodyLSum101/1
  BodyLSum101/1 -> BodyLSum102/2
  BodyDelay102/1 -> b(102)/1, BodyDelay103/1
  b(102)/1 -> BodyLSum102/1
  BodyLSum102/1 -> BodyLSum103/2
  BodyDelay103/1 -> b(103)/1, BodyDelay104/1
  b(103)/1 -> BodyLSum103/1
  BodyLSum103/1 -> BodyLSum104/2
  BodyDelay104/1 -> b(104)/1, BodyDelay105/1
  b(104)/1 -> BodyLSum104/1
  BodyLSum104/1 -> BodyLSum105/2
  BodyDelay105/1 -> b(105)/1, BodyDelay106/1
  b(105)/1 -> BodyLSum105/1
  BodyLSum105/1 -> BodyLSum106/2
  BodyDelay106/1 -> b(106)/1, BodyDelay107/1
  b(106)/1 -> BodyLSum106/1
  BodyLSum106/1 -> BodyLSum107/2
  BodyDelay107/1 -> b(107)/1, BodyDelay108/1
  b(107)/1 -> BodyLSum107/1
  BodyLSum107/1 -> BodyLSum108/2
  BodyDelay108/1 -> b(108)/1, BodyDelay109/1
  b(108)/1 -> BodyLSum108/1
  BodyLSum108/1 -> BodyLSum109/2
  BodyDelay109/1 -> b(109)/1, BodyDelay110/1
  b(109)/1 -> BodyLSum109/1
  BodyLSum109/1 -> BodyLSum110/2
  BodyDelay110/1 -> b(110)/1, BodyDelay111/1
  b(110)/1 -> BodyLSum110/1
  BodyLSum110/1 -> BodyLSum111/2
  BodyDelay111/1 -> b(111)/1, BodyDelay112/1
  b(111)/1 -> BodyLSum111/1
  BodyLSum111/1 -> BodyLSum112/2
  BodyDelay112/1 -> b(112)/1, BodyDelay113/1
  b(112)/1 -> BodyLSum112/1
  BodyLSum112/1 -> BodyLSum113/2
  BodyDelay113/1 -> b(113)/1, BodyDelay114/1
  b(113)/1 -> BodyLSum113/1
  BodyLSum113/1 -> BodyLSum114/2
  BodyDelay114/1 -> b(114)/1, BodyDelay115/1
  b(114)/1 -> BodyLSum114/1
  BodyLSum114/1 -> BodyLSum115/2
  BodyDelay115/1 -> b(115)/1, BodyDelay116/1
  b(115)/1 -> BodyLSum115/1
  BodyLSum115/1 -> BodyLSum116/2
  BodyDelay116/1 -> b(116)/1, BodyDelay117/1
  b(116)/1 -> BodyLSum116/1
  BodyLSum116/1 -> BodyLSum117/2
  BodyDelay117/1 -> b(117)/1, BodyDelay118/1
  b(117)/1 -> BodyLSum117/1
  BodyLSum117/1 -> BodyLSum118/2
  BodyDelay118/1 -> b(118)/1, BodyDelay119/1
  b(118)/1 -> BodyLSum118/1
  BodyLSum118/1 -> BodyLSum119/2
  BodyDelay119/1 -> b(119)/1, BodyDelay120/1
  b(119)/1 -> BodyLSum119/1
  BodyLSum119/1 -> BodyLSum120/2
  BodyDelay120/1 -> b(120)/1, BodyDelay121/1
  b(120)/1 -> BodyLSum120/1
  BodyLSum120/1 -> BodyLSum121/2
  BodyDelay121/1 -> b(121)/1, BodyDelay122/1
  b(121)/1 -> BodyLSum121/1
  BodyLSum121/1 -> BodyLSum122/2
  BodyDelay122/1 -> b(122)/1, BodyDelay123/1
  b(122)/1 -> BodyLSum122/1
  BodyLSum122/1 -> BodyLSum123/2
  BodyDelay123/1 -> b(123)/1, BodyDelay124/1
  b(123)/1 -> BodyLSum123/1
  BodyLSum123/1 -> BodyLSum124/2
  BodyDelay124/1 -> b(124)/1, BodyDelay125/1
  b(124)/1 -> BodyLSum124/1
  BodyLSum124/1 -> BodyLSum125/2
  BodyDelay125/1 -> b(125)/1, BodyDelay126/1
  b(125)/1 -> BodyLSum125/1
  BodyLSum125/1 -> BodyLSum126/2
  BodyDelay126/1 -> b(126)/1, BodyDelay127/1
  b(126)/1 -> BodyLSum126/1
  BodyLSum126/1 -> BodyLSum127/2
  BodyDelay127/1 -> b(127)/1, BodyDelay128/1
  b(127)/1 -> BodyLSum127/1
  BodyLSum127/1 -> BodyLSum128/2
  BodyDelay128/1 -> b(128)/1, BodyDelay129/1
  b(128)/1 -> BodyLSum128/1
  BodyLSum128/1 -> BodyLSum129/2
  BodyDelay129/1 -> b(129)/1, BodyDelay130/1
  b(129)/1 -> BodyLSum129/1
  BodyLSum129/1 -> BodyLSum130/2
  BodyDelay130/1 -> b(130)/1, BodyDelay131/1
  b(130)/1 -> BodyLSum130/1
  BodyLSum130/1 -> BodyLSum131/2
  BodyDelay131/1 -> b(131)/1, BodyDelay132/1
  b(131)/1 -> BodyLSum131/1
  BodyLSum131/1 -> BodyLSum132/2
  BodyDelay132/1 -> b(132)/1, BodyDelay133/1
  b(132)/1 -> BodyLSum132/1
  BodyLSum132/1 -> BodyLSum133/2
  BodyDelay133/1 -> b(133)/1, BodyDelay134/1
  b(133)/1 -> BodyLSum133/1
  BodyLSum133/1 -> BodyLSum134/2
  BodyDelay134/1 -> b(134)/1, BodyDelay135/1
  b(134)/1 -> BodyLSum134/1
  BodyLSum134/1 -> BodyLSum135/2
  BodyDelay135/1 -> b(135)/1, BodyDelay136/1
  b(135)/1 -> BodyLSum135/1
  BodyLSum135/1 -> BodyLSum136/2
  BodyDelay136/1 -> b(136)/1, BodyDelay137/1
  b(136)/1 -> BodyLSum136/1
  BodyLSum136/1 -> BodyLSum137/2
  BodyDelay137/1 -> b(137)/1, BodyDelay138/1
  b(137)/1 -> BodyLSum137/1
  BodyLSum137/1 -> BodyLSum138/2
  BodyDelay138/1 -> b(138)/1, BodyDelay139/1
  b(138)/1 -> BodyLSum138/1
  BodyLSum138/1 -> BodyLSum139/2
  BodyDelay139/1 -> b(139)/1, BodyDelay140/1
  b(139)/1 -> BodyLSum139/1
  BodyLSum139/1 -> BodyLSum140/2
  BodyDelay140/1 -> b(140)/1, BodyDelay141/1
  b(140)/1 -> BodyLSum140/1
  BodyLSum140/1 -> BodyLSum141/2
  BodyDelay141/1 -> b(141)/1, BodyDelay142/1
  b(141)/1 -> BodyLSum141/1
  BodyLSum141/1 -> BodyLSum142/2
  BodyDelay142/1 -> b(142)/1, BodyDelay143/1
  b(142)/1 -> BodyLSum142/1
  BodyLSum142/1 -> BodyLSum143/2
  BodyDelay143/1 -> b(143)/1, BodyDelay144/1
  b(143)/1 -> BodyLSum143/1
  BodyLSum143/1 -> BodyLSum144/2
  BodyDelay144/1 -> b(144)/1, BodyDelay145/1
  b(144)/1 -> BodyLSum144/1
  BodyLSum144/1 -> BodyLSum145/2
  BodyDelay145/1 -> b(145)/1, BodyDelay146/1
  b(145)/1 -> BodyLSum145/1
  BodyLSum145/1 -> BodyLSum146/2
  BodyDelay146/1 -> b(146)/1, BodyDelay147/1
  b(146)/1 -> BodyLSum146/1
  BodyLSum146/1 -> BodyLSum147/2
  BodyDelay147/1 -> b(147)/1, BodyDelay148/1
  b(147)/1 -> BodyLSum147/1
  BodyLSum147/1 -> BodyLSum148/2
  BodyDelay148/1 -> b(148)/1, BodyDelay149/1
  b(148)/1 -> BodyLSum148/1
  BodyLSum148/1 -> BodyLSum149/2
  BodyDelay149/1 -> b(149)/1, BodyDelay150/1
  b(149)/1 -> BodyLSum149/1
  BodyLSum149/1 -> BodyLSum150/2
  BodyDelay150/1 -> b(150)/1, BodyDelay151/1
  b(150)/1 -> BodyLSum150/1
  BodyLSum150/1 -> BodyLSum151/2
  BodyDelay151/1 -> b(151)/1, BodyDelay152/1
  b(151)/1 -> BodyLSum151/1
  BodyLSum151/1 -> BodyLSum152/2
  BodyDelay152/1 -> b(152)/1, BodyDelay153/1
  b(152)/1 -> BodyLSum152/1
  BodyLSum152/1 -> BodyLSum153/2
  BodyDelay153/1 -> b(153)/1, BodyDelay154/1
  b(153)/1 -> BodyLSum153/1
  BodyLSum153/1 -> BodyLSum154/2
  BodyDelay154/1 -> b(154)/1, BodyDelay155/1
  b(154)/1 -> BodyLSum154/1
  BodyLSum154/1 -> BodyLSum155/2
  BodyDelay155/1 -> b(155)/1, BodyDelay156/1
  b(155)/1 -> BodyLSum155/1
  BodyLSum155/1 -> BodyLSum156/2
  BodyDelay156/1 -> b(156)/1, BodyDelay157/1
  b(156)/1 -> BodyLSum156/1
  BodyLSum156/1 -> BodyLSum157/2
  BodyDelay157/1 -> b(157)/1, BodyDelay158/1
  b(157)/1 -> BodyLSum157/1
  BodyLSum157/1 -> BodyLSum158/2
  BodyDelay158/1 -> b(158)/1, BodyDelay159/1
  b(158)/1 -> BodyLSum158/1
  BodyLSum158/1 -> BodyLSum159/2
  BodyDelay159/1 -> b(159)/1, BodyDelay160/1
  b(159)/1 -> BodyLSum159/1
  BodyLSum159/1 -> BodyLSum160/2
  BodyDelay160/1 -> b(160)/1, BodyDelay161/1
  b(160)/1 -> BodyLSum160/1
  BodyLSum160/1 -> BodyLSum161/2
  BodyDelay161/1 -> b(161)/1, BodyDelay162/1
  b(161)/1 -> BodyLSum161/1
  BodyLSum161/1 -> BodyLSum162/2
  BodyDelay162/1 -> b(162)/1, BodyDelay163/1
  b(162)/1 -> BodyLSum162/1
  BodyLSum162/1 -> BodyLSum163/2
  BodyDelay163/1 -> b(163)/1, BodyDelay164/1
  b(163)/1 -> BodyLSum163/1
  BodyLSum163/1 -> BodyLSum164/2
  BodyDelay164/1 -> b(164)/1, BodyDelay165/1
  b(164)/1 -> BodyLSum164/1
  BodyLSum164/1 -> BodyLSum165/2
  BodyDelay165/1 -> b(165)/1, BodyDelay166/1
  b(165)/1 -> BodyLSum165/1
  BodyLSum165/1 -> BodyLSum166/2
  BodyDelay166/1 -> b(166)/1, BodyDelay167/1
  b(166)/1 -> BodyLSum166/1
  BodyLSum166/1 -> BodyLSum167/2
  BodyDelay167/1 -> b(167)/1, BodyDelay168/1
  b(167)/1 -> BodyLSum167/1
  BodyLSum167/1 -> BodyLSum168/2
  BodyDelay168/1 -> b(168)/1, BodyDelay169/1
  b(168)/1 -> BodyLSum168/1
  BodyLSum168/1 -> BodyLSum169/2
  BodyDelay169/1 -> b(169)/1, BodyDelay170/1
  b(169)/1 -> BodyLSum169/1
  BodyLSum169/1 -> BodyLSum170/2
  BodyDelay170/1 -> b(170)/1, BodyDelay171/1
  b(170)/1 -> BodyLSum170/1
  BodyLSum170/1 -> BodyLSum171/2
  BodyDelay171/1 -> b(171)/1, BodyDelay172/1
  b(171)/1 -> BodyLSum171/1
  BodyLSum171/1 -> BodyLSum172/2
  BodyDelay172/1 -> b(172)/1, BodyDelay173/1
  b(172)/1 -> BodyLSum172/1
  BodyLSum172/1 -> BodyLSum173/2
  BodyDelay173/1 -> b(173)/1, BodyDelay174/1
  b(173)/1 -> BodyLSum173/1
  BodyLSum173/1 -> BodyLSum174/2
  BodyDelay174/1 -> b(174)/1, BodyDelay175/1
  b(174)/1 -> BodyLSum174/1
  BodyLSum174/1 -> BodyLSum175/2
  BodyDelay175/1 -> b(175)/1, BodyDelay176/1
  b(175)/1 -> BodyLSum175/1
  BodyLSum175/1 -> BodyLSum176/2
  BodyDelay176/1 -> b(176)/1, BodyDelay177/1
  b(176)/1 -> BodyLSum176/1
  BodyLSum176/1 -> BodyLSum177/2
  BodyDelay177/1 -> b(177)/1, BodyDelay178/1
  b(177)/1 -> BodyLSum177/1
  BodyLSum177/1 -> BodyLSum178/2
  BodyDelay178/1 -> b(178)/1, BodyDelay179/1
  b(178)/1 -> BodyLSum178/1
  BodyLSum178/1 -> BodyLSum179/2
  BodyDelay179/1 -> b(179)/1, BodyDelay180/1
  b(179)/1 -> BodyLSum179/1
  BodyLSum179/1 -> BodyLSum180/2
  BodyDelay180/1 -> b(180)/1, BodyDelay181/1
  b(180)/1 -> BodyLSum180/1
  BodyLSum180/1 -> BodyLSum181/2
  BodyDelay181/1 -> b(181)/1, BodyDelay182/1
  b(181)/1 -> BodyLSum181/1
  BodyLSum181/1 -> BodyLSum182/2
  BodyDelay182/1 -> b(182)/1, BodyDelay183/1
  b(182)/1 -> BodyLSum182/1
  BodyLSum182/1 -> BodyLSum183/2
  BodyDelay183/1 -> b(183)/1, BodyDelay184/1
  b(183)/1 -> BodyLSum183/1
  BodyLSum183/1 -> BodyLSum184/2
  BodyDelay184/1 -> b(184)/1, BodyDelay185/1
  b(184)/1 -> BodyLSum184/1
  BodyLSum184/1 -> BodyLSum185/2
  BodyDelay185/1 -> b(185)/1, BodyDelay186/1
  b(185)/1 -> BodyLSum185/1
  BodyLSum185/1 -> BodyLSum186/2
  BodyDelay186/1 -> b(186)/1, BodyDelay187/1
  b(186)/1 -> BodyLSum186/1
  BodyLSum186/1 -> BodyLSum187/2
  BodyDelay187/1 -> b(187)/1, BodyDelay188/1
  b(187)/1 -> BodyLSum187/1
  BodyLSum187/1 -> BodyLSum188/2
  BodyDelay188/1 -> b(188)/1, BodyDelay189/1
  b(188)/1 -> BodyLSum188/1
  BodyLSum188/1 -> BodyLSum189/2
  BodyDelay189/1 -> b(189)/1, BodyDelay190/1
  b(189)/1 -> BodyLSum189/1
  BodyLSum189/1 -> BodyLSum190/2
  BodyDelay190/1 -> b(190)/1, BodyDelay191/1
  b(190)/1 -> BodyLSum190/1
  BodyLSum190/1 -> BodyLSum191/2
  BodyDelay191/1 -> b(191)/1, BodyDelay192/1
  b(191)/1 -> BodyLSum191/1
  BodyLSum191/1 -> BodyLSum192/2
  BodyDelay192/1 -> b(192)/1, BodyDelay193/1
  b(192)/1 -> BodyLSum192/1
  BodyLSum192/1 -> BodyLSum193/2
  BodyDelay193/1 -> b(193)/1, BodyDelay194/1
  b(193)/1 -> BodyLSum193/1
  BodyLSum193/1 -> BodyLSum194/2
  BodyDelay194/1 -> b(194)/1, BodyDelay195/1
  b(194)/1 -> BodyLSum194/1
  BodyLSum194/1 -> BodyLSum195/2
  BodyDelay195/1 -> b(195)/1, BodyDelay196/1
  b(195)/1 -> BodyLSum195/1
  BodyLSum195/1 -> BodyLSum196/2
  BodyDelay196/1 -> b(196)/1, BodyDelay197/1
  b(196)/1 -> BodyLSum196/1
  BodyLSum196/1 -> BodyLSum197/2
  BodyDelay197/1 -> b(197)/1, BodyDelay198/1
  b(197)/1 -> BodyLSum197/1
  BodyLSum197/1 -> BodyLSum198/2
  BodyDelay198/1 -> b(198)/1, BodyDelay199/1
  b(198)/1 -> BodyLSum198/1
  BodyLSum198/1 -> BodyLSum199/2
  BodyDelay199/1 -> b(199)/1, BodyDelay200/1
  b(199)/1 -> BodyLSum199/1
  BodyLSum199/1 -> BodyLSum200/2
  BodyDelay200/1 -> b(200)/1, BodyDelay201/1
  b(200)/1 -> BodyLSum200/1
  BodyLSum200/1 -> BodyLSum201/2
  BodyDelay201/1 -> b(201)/1, BodyDelay202/1
  b(201)/1 -> BodyLSum201/1
  BodyLSum201/1 -> BodyLSum202/2
  BodyDelay202/1 -> b(202)/1, BodyDelay203/1
  b(202)/1 -> BodyLSum202/1
  BodyLSum202/1 -> BodyLSum203/2
  BodyDelay203/1 -> b(203)/1, BodyDelay204/1
  b(203)/1 -> BodyLSum203/1
  BodyLSum203/1 -> BodyLSum204/2
  BodyDelay204/1 -> b(204)/1, BodyDelay205/1
  b(204)/1 -> BodyLSum204/1
  BodyLSum204/1 -> BodyLSum205/2
  BodyDelay205/1 -> b(205)/1, BodyDelay206/1
  b(205)/1 -> BodyLSum205/1
  BodyLSum205/1 -> BodyLSum206/2
  BodyDelay206/1 -> b(206)/1, BodyDelay207/1
  b(206)/1 -> BodyLSum206/1
  BodyLSum206/1 -> BodyLSum207/2
  BodyDelay207/1 -> b(207)/1, BodyDelay208/1
  b(207)/1 -> BodyLSum207/1
  BodyLSum207/1 -> BodyLSum208/2
  BodyDelay208/1 -> b(208)/1, BodyDelay209/1
  b(208)/1 -> BodyLSum208/1
  BodyLSum208/1 -> BodyLSum209/2
  BodyDelay209/1 -> b(209)/1, BodyDelay210/1
  b(209)/1 -> BodyLSum209/1
  BodyLSum209/1 -> BodyLSum210/2
  BodyDelay210/1 -> b(210)/1, BodyDelay211/1
  b(210)/1 -> BodyLSum210/1
  BodyLSum210/1 -> BodyLSum211/2
  BodyDelay211/1 -> b(211)/1, BodyDelay212/1
  b(211)/1 -> BodyLSum211/1
  BodyLSum211/1 -> BodyLSum212/2
  BodyDelay212/1 -> b(212)/1, BodyDelay213/1
  b(212)/1 -> BodyLSum212/1
  BodyLSum212/1 -> BodyLSum213/2
  BodyDelay213/1 -> b(213)/1, BodyDelay214/1
  b(213)/1 -> BodyLSum213/1
  BodyLSum213/1 -> BodyLSum214/2
  BodyDelay214/1 -> b(214)/1, BodyDelay215/1
  b(214)/1 -> BodyLSum214/1
  BodyLSum214/1 -> BodyLSum215/2
  BodyDelay215/1 -> b(215)/1, BodyDelay216/1
  b(215)/1 -> BodyLSum215/1
  BodyLSum215/1 -> BodyLSum216/2
  BodyDelay216/1 -> b(216)/1, BodyDelay217/1
  b(216)/1 -> BodyLSum216/1
  BodyLSum216/1 -> BodyLSum217/2
  BodyDelay217/1 -> b(217)/1, BodyDelay218/1
  b(217)/1 -> BodyLSum217/1
  BodyLSum217/1 -> BodyLSum218/2
  BodyDelay218/1 -> b(218)/1, BodyDelay219/1
  b(218)/1 -> BodyLSum218/1
  BodyLSum218/1 -> BodyLSum219/2
  BodyDelay219/1 -> b(219)/1, BodyDelay220/1
  b(219)/1 -> BodyLSum219/1
  BodyLSum219/1 -> BodyLSum220/2
  BodyDelay220/1 -> b(220)/1, BodyDelay221/1
  b(220)/1 -> BodyLSum220/1
  BodyLSum220/1 -> BodyLSum221/2
  BodyDelay221/1 -> b(221)/1, BodyDelay222/1
  b(221)/1 -> BodyLSum221/1
  BodyLSum221/1 -> BodyLSum222/2
  BodyDelay222/1 -> b(222)/1, BodyDelay223/1
  b(222)/1 -> BodyLSum222/1
  BodyLSum222/1 -> BodyLSum223/2
  BodyDelay223/1 -> b(223)/1, BodyDelay224/1
  b(223)/1 -> BodyLSum223/1
  BodyLSum223/1 -> BodyLSum224/2
  BodyDelay224/1 -> b(224)/1, BodyDelay225/1
  b(224)/1 -> BodyLSum224/1
  BodyLSum224/1 -> BodyLSum225/2
  BodyDelay225/1 -> b(225)/1, BodyDelay226/1
  b(225)/1 -> BodyLSum225/1
  BodyLSum225/1 -> BodyLSum226/2
  BodyDelay226/1 -> b(226)/1, BodyDelay227/1
  b(226)/1 -> BodyLSum226/1
  BodyLSum226/1 -> BodyLSum227/2
  BodyDelay227/1 -> b(227)/1, BodyDelay228/1
  b(227)/1 -> BodyLSum227/1
  BodyLSum227/1 -> BodyLSum228/2
  BodyDelay228/1 -> b(228)/1, BodyDelay229/1
  b(228)/1 -> BodyLSum228/1
  BodyLSum228/1 -> BodyLSum229/2
  BodyDelay229/1 -> b(229)/1, BodyDelay230/1
  b(229)/1 -> BodyLSum229/1
  BodyLSum229/1 -> BodyLSum230/2
  BodyDelay230/1 -> b(230)/1, BodyDelay231/1
  b(230)/1 -> BodyLSum230/1
  BodyLSum230/1 -> BodyLSum231/2
  BodyDelay231/1 -> b(231)/1, BodyDelay232/1
  b(231)/1 -> BodyLSum231/1
  BodyLSum231/1 -> BodyLSum232/2
  BodyDelay232/1 -> b(232)/1, BodyDelay233/1
  b(232)/1 -> BodyLSum232/1
  BodyLSum232/1 -> BodyLSum233/2
  BodyDelay233/1 -> b(233)/1, BodyDelay234/1
  b(233)/1 -> BodyLSum233/1
  BodyLSum233/1 -> BodyLSum234/2
  BodyDelay234/1 -> b(234)/1, BodyDelay235/1
  b(234)/1 -> BodyLSum234/1
  BodyLSum234/1 -> BodyLSum235/2
  BodyDelay235/1 -> b(235)/1, BodyDelay236/1
  b(235)/1 -> BodyLSum235/1
  BodyLSum235/1 -> BodyLSum236/2
  BodyDelay236/1 -> b(236)/1, BodyDelay237/1
  b(236)/1 -> BodyLSum236/1
  BodyLSum236/1 -> BodyLSum237/2
  BodyDelay237/1 -> b(237)/1, BodyDelay238/1
  b(237)/1 -> BodyLSum237/1
  BodyLSum237/1 -> BodyLSum238/2
  BodyDelay238/1 -> b(238)/1, BodyDelay239/1
  b(238)/1 -> BodyLSum238/1
  BodyLSum238/1 -> BodyLSum239/2
  BodyDelay239/1 -> b(239)/1, BodyDelay240/1
  b(239)/1 -> BodyLSum239/1
  BodyLSum239/1 -> BodyLSum240/2
  BodyDelay240/1 -> b(240)/1, BodyDelay241/1
  b(240)/1 -> BodyLSum240/1
  BodyLSum240/1 -> BodyLSum241/2
  BodyDelay241/1 -> b(241)/1, BodyDelay242/1
  b(241)/1 -> BodyLSum241/1
  BodyLSum241/1 -> BodyLSum242/2
  BodyDelay242/1 -> b(242)/1, BodyDelay243/1
  b(242)/1 -> BodyLSum242/1
  BodyLSum242/1 -> BodyLSum243/2
  BodyDelay243/1 -> b(243)/1, BodyDelay244/1
  b(243)/1 -> BodyLSum243/1
  BodyLSum243/1 -> BodyLSum244/2
  BodyDelay244/1 -> b(244)/1, BodyDelay245/1
  b(244)/1 -> BodyLSum244/1
  BodyLSum244/1 -> BodyLSum245/2
  BodyDelay245/1 -> b(245)/1, BodyDelay246/1
  b(245)/1 -> BodyLSum245/1
  BodyLSum245/1 -> BodyLSum246/2
  BodyDelay246/1 -> b(246)/1, BodyDelay247/1
  b(246)/1 -> BodyLSum246/1
  BodyLSum246/1 -> BodyLSum247/2
  BodyDelay247/1 -> b(247)/1, BodyDelay248/1
  b(247)/1 -> BodyLSum247/1
  BodyLSum247/1 -> BodyLSum248/2
  BodyDelay248/1 -> b(248)/1, BodyDelay249/1
  b(248)/1 -> BodyLSum248/1
  BodyLSum248/1 -> BodyLSum249/2
  BodyDelay249/1 -> b(249)/1, BodyDelay250/1
  b(249)/1 -> BodyLSum249/1
  BodyLSum249/1 -> BodyLSum250/2
  BodyDelay250/1 -> b(250)/1, BodyDelay251/1
  b(250)/1 -> BodyLSum250/1
  BodyLSum250/1 -> BodyLSum251/2
  BodyDelay251/1 -> b(251)/1, BodyDelay252/1
  b(251)/1 -> BodyLSum251/1
  BodyLSum251/1 -> BodyLSum252/2
  BodyDelay252/1 -> b(252)/1, BodyDelay253/1
  b(252)/1 -> BodyLSum252/1
  BodyLSum252/1 -> BodyLSum253/2
  BodyDelay253/1 -> b(253)/1, BodyDelay254/1
  b(253)/1 -> BodyLSum253/1
  BodyLSum253/1 -> BodyLSum254/2
  BodyDelay254/1 -> b(254)/1, BodyDelay255/1
  b(254)/1 -> BodyLSum254/1
  BodyLSum254/1 -> BodyLSum255/2
  BodyDelay255/1 -> b(255)/1, BodyDelay256/1
  b(255)/1 -> BodyLSum255/1
  BodyLSum255/1 -> BodyLSum256/2
  BodyDelay256/1 -> b(256)/1, BodyDelay257/1
  b(256)/1 -> BodyLSum256/1
  BodyLSum256/1 -> BodyLSum257/2
  BodyDelay257/1 -> b(257)/1, BodyDelay258/1
  b(257)/1 -> BodyLSum257/1
  BodyLSum257/1 -> BodyLSum258/2
  BodyDelay258/1 -> b(258)/1, BodyDelay259/1
  b(258)/1 -> BodyLSum258/1
  BodyLSum258/1 -> BodyLSum259/2
  BodyDelay259/1 -> b(259)/1, BodyDelay260/1
  b(259)/1 -> BodyLSum259/1
  BodyLSum259/1 -> BodyLSum260/1
  BodyDelay260/1 -> b(260)/1
  b(260)/1 -> BodyLSum260/2
  BodyLSum260/1 -> Output/1
